simulink model "FullFMS_2026_02_25_V0_4_4"  (R2026a)
settings: Solver=FixedStepAuto  StopTime=inf  FixedStep=0.01  MaxStep=0.01  RelTol=1e-2
PreLoadFcn:
  | load("BUS_CONFIG.mat")
libraries: opcualib x8
(part 3 of 5)

== stateflow chart FullFMS_2026_02_25_V0_4_4/Chart ==
  state Variable_Declaration
    state VarDeclaration_20
      entry:
      %Actuators
      Actuators_20.F_22_Led_On;
      Actuators_20.F_22_Led_Off;
      Actuators_20.F_22_Conveyor;
      Actuators_20.F_24_Release_FB;
      Actuators_20.F_25_Release_FB;
      Actuators_20.F_26_Release_FB;
      Actuators_20.F_27_Release_FB;
      Actuators_20.F_28_Release_FB;
      Actuators_20.F_29_Release_FB;
      %Control
      Control_20.C_24_CartDel;
      Control_20.C_24_CRoute_Out;
      Control_20.C_24_Request;
      Control_20.C_24_CRoute_In;
      Control_20.C_25_CartDel;
      Control_20.C_25_CRoute_Out;
      Control_20.C_25_Request;
      Control_20.C_25_CRoute_In;
      Control_20.C_26_CartDel;
      Control_20.C_26_CRoute_Out;
      Control_20.C_26_Request;
      Control_20.C_26_CRoute_In;
      Control_20.C_27_CartDel;
      Control_20.C_27_CRoute_Out;
      Control_20.C_27_Request;
      Control_20.C_27_CRoute_In;
      Control_20.C_28_CartDel;
      Control_20.C_28_CRoute_Out;
      Control_20.C_28_Request;
      Control_20.C_28_CRoute_In;
      Control_20.C_29_CartDel;
      Control_20.C_29_CRoute_Out;
      Control_20.C_29_Request;
      Control_20.C_29_CRoute_In;
      %Sensors
      Sensors_20.O_20_On;
      Sensors_20.O_20_Off;
      Sensors_20.O_20_Controler_On;
      Sensors_20.O_24_Cart_Stat;
      Sensors_20.O_24_Cart_Next;
      Sensors_20.O_24_Optic;
      Sensors_20.O_24_Count;
      Sensors_20.O_24_Pist_Bck;
      Sensors_20.O_25_Cart_Stat;
      Sensors_20.O_25_Cart_Next;
      Sensors_20.O_25_Optic;
      Sensors_20.O_25_Count;
      Sensors_20.O_25_Pist_Bck;
      Sensors_20.O_26_Cart_Stat;
      Sensors_20.O_26_Cart_Next;
      Sensors_20.O_26_Optic;
      Sensors_20.O_26_Count;
      Sensors_20.O_26_Pist_Bck;
      Sensors_20.O_27_Cart_Stat;
      Sensors_20.O_27_Cart_Next;
      Sensors_20.O_27_Optic;
      Sensors_20.O_27_Count;
      Sensors_20.O_27_Pist_Bck;
      Sensors_20.O_28_Cart_Stat;
      Sensors_20.O_28_Cart_Next;
      Sensors_20.O_28_Optic;
      Sensors_20.O_28_Count;
      Sensors_20.O_28_Pist_Bck;
      Sensors_20.O_29_Cart_Stat;
      Sensors_20.O_29_Cart_Next;
      Sensors_20.O_29_Optic;
      Sensors_20.O_29_Count;
      Sensors_20.O_29_Pist_Bck;
    state VarDeclaration_30
      entry:
      %Actuators
      Actuators_30.F_33_Led_Start;
      Actuators_30.F_33_Led_Reset;
      Actuators_30.F_33_Led_Extra1;
      Actuators_30.F_33_Led_Extra2;
      Actuators_30.F_33_Spring_Cyl;
      Actuators_30.F_33_Cover_Cyl;
      %AS-i
      AS_i_30.A_34_Request;
      AS_i_30.A_34_No_Cart;
      AS_i_30.A_34_Cart_Full;
      AS_i_30.A_34_CRoute_Out;
      AS_i_30.A_32_RoboCartID;
      AS_i_30.A_34_Cart_Stat;
      AS_i_30.A_34_Cart_Next;
      AS_i_30.A_34_Optic;
      AS_i_30.A_34_Count;
      AS_i_30.A_34_Pist_Bck;
      AS_i_30.A_34_Release_FB;
      AS_i_30.A_34_CRoute_In;
      %Control
      Control_30.C_30_Robot1;
      Control_30.C_30_Robot2;
      Control_30.C_35_Part_Del;
      %Sensors
      Sensors_30.O_31_Start;
      Sensors_30.O_31_Stop;
      Sensors_30.O_31_Reset;
      Sensors_30.O_31_Part_in_Claw;
      Sensors_30.O_31_Orientation;
      Sensors_30.O_32_Sp_Cyl_Bck;
      Sensors_30.O_32_Sp_Cyl_Fwd;
      Sensors_30.O_32_Co_Cyl_Bck;
      Sensors_30.O_32_Co_Cyl_Fwd;
      Sensors_30.O_32_Sp_PickUp;
      Sensors_30.O_32_Co_PickUp;
      Sensors_30.O_32_CoMag_Empty;
    state VarDeclaration_40
      entry:
      %Actuators
      Actuators_40.F_43_Led_Start;
      Actuators_40.F_43_Led_Reset;
      Actuators_40.F_43_Led_Extra1;
      Actuators_40.F_43_Led_Extra2;
      Actuators_40.F_43_Panel_O4;
      Actuators_40.F_43_Panel_O5;
      Actuators_40.F_43_Panel_O6;
      Actuators_40.F_43_Panel_O7;
      %AS-i
      AS_i_40.A_44_Request;
      AS_i_40.A_44_No_Cart;
      AS_i_40.A_44_Cart_Full;
      AS_i_40.A_44_CRoute_Out;
      AS_i_40.A_43_StorCartID;
      AS_i_40.A_44_Cart_Stat;
      AS_i_40.A_44_Cart_Next;
      AS_i_40.A_44_Optic;
      AS_i_40.A_44_Count;
      AS_i_40.A_44_Pist_Bck;
      AS_i_40.A_44_Release_FB;
      AS_i_40.A_44_CRoute_In;
      %Control
      Control_40.C_45_Initialization;
      Control_40.C_42_Profibus;
      Control_40.C_45_Start;
      Control_40.C_45_StorePart;
      Control_40.C_45_RetrievePart;
      %Sensors
      Sensors_40.O_41_Start;
      Sensors_40.O_41_Stop;
      Sensors_40.O_41_Key_Pos;
      Sensors_40.O_41_Reset;
      Sensors_40.O_41_Panel_I4;
      Sensors_40.O_41_Panel_I5;
      Sensors_40.O_41_Panel_I6;
      Sensors_40.O_41_Panel_I7;
    state VarDeclaration_50
      entry:
      %Actuators
      Actuators_50.F_52_Claw_2_Del;
      Actuators_50.F_52_Claw_2_Cart;
      Actuators_50.F_52_Claw_Down;
      Actuators_50.F_52_Close_Claw;
      Actuators_50.F_53_Led_Start;
      Actuators_50.F_53_Led_Reset;
      Actuators_50.F_53_Led_Extra1;
      Actuators_50.F_53_Led_Extra2;
      Actuators_50.F_53_Panel_O4;
      Actuators_50.F_53_Panel_O5;
      Actuators_50.F_53_Panel_O6;
      Actuators_50.F_53_Panel_O7;
      %AS-i
      AS_i_50.A_54_Request;
      AS_i_50.A_54_No_Cart;
      AS_i_50.A_54_Cart_Full;
      AS_i_50.A_54_CRoute_Out;
      AS_i_50.A_53_SortCartID;
      AS_i_50.A_54_Cart_Stat;
      AS_i_50.A_54_Cart_Next;
      AS_i_50.A_54_Optic;
      AS_i_50.A_54_Count;
      AS_i_50.A_54_Pist_Bck;
      AS_i_50.A_54_Release_FB;
      AS_i_50.A_54_CRoute_In;
      %Control
      Control_50.C_55_Initialization;
      Control_50.C_55_PD_Sort;
      Control_50.C_52_Profibus;
      Control_50.C_55_Start;
      Control_50.C_55_Cart2Del;
      %Sensors
      Sensors_50.O_50_Part_Reserve;
      Sensors_50.O_50_Claw_Cart;
      Sensors_50.O_50_Claw_Del;
      Sensors_50.O_50_Claw_Reserve;
      Sensors_50.O_50_Claw_Low;
      Sensors_50.O_50_Claw_High;
      Sensors_50.O_50_Part_in_Claw;
      Sensors_50.O_51_Start;
      Sensors_50.O_51_Stop;
      Sensors_50.O_51_Key_Pos;
      Sensors_50.O_51_Reset;
      Sensors_50.O_51_Panel_I4;
      Sensors_50.O_51_Panel_I5;
      Sensors_50.O_51_Panel_I6;
      Sensors_50.O_51_Panel_I7;
    state VarDeclaration_60
      entry:
      %Actuators
      Actuators_60.F_62_Conveyor;
      Actuators_60.F_62_P1;
      Actuators_60.F_62_P2;
      Actuators_60.F_62_Identify;
      Actuators_60.F_63_Led_Start;
      Actuators_60.F_63_Led_Reset;
      Actuators_60.F_63_Led_Extra1;
      Actuators_60.F_63_Led_Extra2;
      Actuators_60.F_63_Panel_O4;
      Actuators_60.F_63_Panel_O5;
      Actuators_60.F_63_Panel_O6;
      Actuators_60.F_63_Panel_O7;
      %Control
      Control_60.C_65_Initialization;
      Control_60.C_65_ID_1;
      Control_60.C_65_ID_2;
      Control_60.C_65_Part_Sorted;
      Control_60.C_62_Profibus;
      Control_60.C_65_RBS_Output;
      Control_60.C_65_RSB_Output;
      Control_60.C_65_BRS_Output;
      Control_60.C_65_BSR_Output;
      Control_60.C_65_SRB_Output;
      Control_60.C_65_SBR_Output;
      %Sensors
      Sensors_60.O_60_SPart;
      Sensors_60.O_60_SInd;
      Sensors_60.O_60_SPhoto;
      Sensors_60.O_60_Part_Pass;
      Sensors_60.O_60_SL1_Bck;
      Sensors_60.O_60_SL1_Fwd;
      Sensors_60.O_60_SL2_Bck;
      Sensors_60.O_60_SL2_Fwd;
      Sensors_60.O_61_Start;
      Sensors_60.O_61_Stop;
      Sensors_60.O_61_Key_Pos;
      Sensors_60.O_61_Reset;
      Sensors_60.O_61_Panel_I4;
      Sensors_60.O_61_Panel_I5;
      Sensors_60.O_61_Panel_I6;
      Sensors_60.O_61_Panel_I7;
    state VarDeclaration_70
      entry:
      %Actuators
      Actuators_70.F_72_Elev_Down;
      Actuators_70.F_72_Elev_Up;
      Actuators_70.F_72_Eject_Part;
      Actuators_70.F_72_Air_On;
      Actuators_70.F_73_Led_Start;
      Actuators_70.F_73_Led_Reset;
      Actuators_70.F_73_Led_Extra1;
      Actuators_70.F_73_Led_Extra2;
      Actuators_70.F_73_Panel_O4;
      Actuators_70.F_73_Panel_O5;
      Actuators_70.F_73_Panel_O6;
      Actuators_70.F_73_Panel_O7;
      %AS-i
      AS_i_70.A_74_Request;
      AS_i_70.A_74_No_Cart;
      AS_i_70.A_74_Cart_Full;
      AS_i_70.A_74_CRoute_Out;
      AS_i_70.A_74_CRoute_In80;
      AS_i_70.A_73_TestCartID;
      AS_i_70.A_74_Cart_Stat;
      AS_i_70.A_74_Cart_Next;
      AS_i_70.A_74_Optic;
      AS_i_70.A_74_Count;
      AS_i_70.A_74_Pist_Bck;
      AS_i_70.A_74_Release_FB;
      AS_i_70.A_74_CRoute_In;
      %Control
      Control_70.C_75_Initialization;
      Control_70.C_75_ID_Delivery1;
      Control_70.C_75_ID_Delivery2;
      Control_70.C_75_Part_Del;
      Control_70.C_75_RQ_Part_Del;
      Control_70.C_75_RQ_Wrong;
      Control_70.C_75_Identified80;
      Control_70.C_75_Requested80;
      Control_70.C_72_Profibus;
      Control_70.C_75_RQ_Delivery1;
      Control_70.C_75_RQ_Delivery2;
      Control_70.C_75_Identified;
      Control_70.C_75_Requested;
      %Sensors
      Sensors_70.O_70_SInductive;
      Sensors_70.O_70_SPart;
      Sensors_70.O_70_SStation;
      Sensors_70.O_70_SPart_Height;
      Sensors_70.O_70_Elev_High;
      Sensors_70.O_70_Elev_Low;
      Sensors_70.O_70_Pist_Bck;
      Sensors_70.O_71_Start;
      Sensors_70.O_71_Stop;
      Sensors_70.O_71_Key_Pos;
      Sensors_70.O_71_Reset;
      Sensors_70.O_71_Panel_I4;
      Sensors_70.O_71_Panel_I5;
      Sensors_70.O_71_Panel_I6;
      Sensors_70.O_71_Panel_I7;
    state VarDeclaration_80
      entry:
      %Actuators
      Actuators_80.F_82_Pist_Adv;
      Actuators_80.F_82_Suction_On;
      Actuators_80.F_82_Suction_Off;
      Actuators_80.F_82_Arm_2_Del;
      Actuators_80.F_82_Arm_2_Mag;
      Actuators_80.F_83_Led_Start;
      Actuators_80.F_83_Led_Reset;
      Actuators_80.F_83_Led_Extra1;
      Actuators_80.F_83_Led_Extra2;
      Actuators_80.F_83_Panel_O4;
      Actuators_80.F_83_Panel_O5;
      Actuators_80.F_83_Panel_O6;
      Actuators_80.F_83_Panel_O7;
      %Control
      Control_80.C_85_Initialization;
      Control_80.C_85_Part_Del;
      Control_80.C_85_Part_Mag;
      Control_80.C_86_Mag_Parts;
      Control_80.C_87_RQ_MParts;
      Control_80.C_82_Profibus;
      Control_80.C_83_RQ_Parts;
      Control_80.C_85_Start;
      Control_80.C_85_Single;
      Control_80.C_85_Continuous;
      Control_80.C_85_Counted;
      %Sensors
      Sensors_80.O_80_Mag_Full;
      Sensors_80.O_80_Pist_Bck;
      Sensors_80.O_80_Pist_Fwd;
      Sensors_80.O_80_Part_Stuck;
      Sensors_80.O_80_Arm_Mag;
      Sensors_80.O_80_Arm_Del;
      Sensors_80.O_80_Mag_Empty;
      Sensors_80.O_81_Start;
      Sensors_80.O_81_Stop;,
      Sensors_80.O_81_Key_Pos;
      Sensors_80.O_81_Reset;
      Sensors_80.O_81_Panel_I4;
      Sensors_80.O_81_Panel_I5;
      Sensors_80.O_81_Panel_I6;
      Sensors_80.O_81_Panel_I7;
    state VarDeclaration_90
      entry:
      %Actuators
      Actuators_90.F_92_Claw_2_Cart;
      Actuators_90.F_92_Claw_2_Del;
      Actuators_90.F_92_Claw_Down;
      Actuators_90.F_92_Close_Claw;
      Actuators_90.F_93_Led_Start;
      Actuators_90.F_93_Led_Reset;
      Actuators_90.F_93_Led_Extra1;
      Actuators_90.F_93_Led_Extra2;
      Actuators_90.F_93_Panel_O4;
      Actuators_90.F_93_Panel_O5;
      Actuators_90.F_93_Panel_O6;
      Actuators_90.F_93_Panel_O7;
      %AS-i
      AS_i_90.A_94_Request;
      AS_i_90.A_94_No_Cart;
      AS_i_90.A_94_Cart_Full;
      AS_i_90.A_94_CRoute_Out;
      AS_i_90.A_93_ProcCartID;
      AS_i_90.A_94_Cart_Stat;
      AS_i_90.A_94_Cart_Next;
      AS_i_90.A_94_Optic;
      AS_i_90.A_94_Count;
      AS_i_90.A_94_Pist_Bck;
      AS_i_90.A_94_Release_FB;
      AS_i_90.A_94_CRoute_In;
      %Control
      Control_90.C_95_Initialization;
      Control_90.C_95_PD_Proc;
      Control_90.C_95_PD_Cart;
      Control_90.C_92_Profibus;
      Control_90.C_95_Start;
      Control_90.C_95_Cart2Del;
      Control_90.C_95_Del2Cart;
      %Sensors
      Sensors_90.O_90_Part_Reserve;
      Sensors_90.O_90_Claw_Del;
      Sensors_90.O_90_Claw_Cart;
      Sensors_90.O_90_Claw_Reserve;
      Sensors_90.O_90_Claw_Low;
      Sensors_90.O_90_Claw_High;
      Sensors_90.O_90_Part_in_Claw;
      Sensors_90.O_91_Start;
      Sensors_90.O_91_Stop;
      Sensors_90.O_91_Key_Pos;
      Sensors_90.O_91_Reset;
      Sensors_90.O_91_Panel_I4;
      Sensors_90.O_91_Panel_I5;
      Sensors_90.O_91_Panel_I6;
      Sensors_90.O_91_Panel_I7;
    state VarDeclaration_100
      entry:
      %Actuators
      Actuators_100.F_102_Drill_On;
      Actuators_100.F_102_RT_On;
      Actuators_100.F_102_Drill_Down;
      Actuators_100.F_102_Drill_Up;
      Actuators_100.F_102_Drill_Pin;
      Actuators_100.F_102_Test_Pin;
      Actuators_100.F_103_Led_Start;
      Actuators_100.F_103_Led_Reset;
      Actuators_100.F_103_Led_Extra1;
      Actuators_100.F_103_Led_Extra2;
      Actuators_100.F_103_Panel_O4;
      Actuators_100.F_103_Panel_O5;
      Actuators_100.F_103_Panel_O6;
      Actuators_100.F_103_Panel_O7;
      %Control
      Control_100.C_105_Initialization;
      Control_100.C_105_Part_ready;
      Control_100.C_105_Test_Ok;
      Control_100.C_105_Test_Fail;
      Control_100.C_106_RT_Counter;
      Control_100.C_102_Profibus;
      Control_100.C_103_RQ_Turns;
      Control_100.C_105_Start;
      Control_100.C_105_Test;
      Control_100.C_105_TestDrill;
      Control_100.C_105_Rotation;
      %Sensors
      Sensors_100.O_100_PInit_Pos;
      Sensors_100.O_100_PDrill_Pos;
      Sensors_100.O_100_PTest_Pos;
      Sensors_100.O_100_SDrill_High;
      Sensors_100.O_100_SDrill_Low;
      Sensors_100.O_100_RT_Sensor;
      Sensors_100.O_100_PTest_Ok;
      Sensors_100.O_101_Start;
      Sensors_100.O_101_Stop;
      Sensors_100.O_101_Key_Pos;
      Sensors_100.O_101_Reset;
      Sensors_100.O_101_Panel_I4;
      Sensors_100.O_101_Panel_I5;
      Sensors_100.O_101_Panel_I6;
      Sensors_100.O_101_Panel_I7;
    (default) -> VarDeclaration_20
    VarDeclaration_60 -> VarDeclaration_70
    VarDeclaration_30 -> VarDeclaration_40
    VarDeclaration_40 -> VarDeclaration_50
    VarDeclaration_70 -> VarDeclaration_80
    VarDeclaration_80 -> VarDeclaration_90
    VarDeclaration_50 -> VarDeclaration_60
    VarDeclaration_90 -> VarDeclaration_100
    VarDeclaration_20 -> VarDeclaration_30
  note: Sorting [60]
  state BRS Output
    state ArmToMagazine1
      entry:
      Status2c_14 = false;
      during:
      Actuators_80.F_82_Suction_Off;
      Actuators_80.F_82_Arm_2_Mag;
      Actuators_80.F_83_Led_Extra1;
      Control_80.C_85_Part_Del;
      if ~Actuators_80.F_82_Suction_Off && ...
      Actuators_80.F_82_Arm_2_Mag && ...
      Actuators_80.F_83_Led_Extra1 && ...
      Control_80.C_85_Part_Del
      Status2c_14 = true;
      else
      Status2c_14 = false;
      end
    state ArmCloseDeliver3
      entry:
      Status2c_15 = false;
      during:
      Sensors_70.O_70_SStation;
      if Sensors_70.O_70_SStation
      Status2c_15 = true;
      else
      Status2c_15 = false;
      end
    state ArmArrives_Finish
      entry:
      Status2c_16 = false;
      during:
      Actuators_80.F_82_Arm_2_Mag;
      if ~Actuators_80.F_82_Arm_2_Mag;
      Status2c_16 = true;
      else
      Status2c_16 = false;
      end
    state ArmToMagazine
      entry:
      Status2c_8 = false;
      during:
      Actuators_80.F_82_Arm_2_Mag;
      if Actuators_80.F_82_Arm_2_Mag
      Status2c_8 = true;
      else
      Status2c_8 = false;
      end
    state ArmCloseDeliver1
      entry:
      Status2c_9 = false;
      during:
      Sensors_70.O_70_SStation;
      if Sensors_70.O_70_SStation
      Status2c_9 = true;
      else
      Status2c_9 = false;
      end
    state ArmArrives_PicksPart
      entry:
      Status2c_10 = false;
      during:
      Actuators_80.F_82_Suction_On;
      Actuators_80.F_82_Arm_2_Mag;
      if Actuators_80.F_82_Suction_On && ...
      ~Actuators_80.F_82_Arm_2_Mag
      Status2c_10 = true;
      else
      Status2c_10 = false;
      end
    state ArmToDelivery1
      entry:
      Status2c_11 = false;
      during:
      Actuators_80.F_82_Arm_2_Del
      if Actuators_80.F_82_Arm_2_Del
      Status2c_11 = true;
      else
      Status2c_11 = false;
      end
    state ArmCloseDelivery2
      entry:
      Status2c_12 = false;
      during:
      Sensors_70.O_70_SStation;
      if Sensors_70.O_70_SStation
      Status2c_12 = true;
      else
      Status2c_12 = false;
      end
    state ArmArrives_DeliversPart
      entry:
      Status2c_13 = false;
      during:
      Actuators_80.F_82_Suction_On;
      Actuators_80.F_82_Suction_Off;
      Actuators_80.F_82_Arm_2_Del;
      if ~Actuators_80.F_82_Suction_On && ...
      Actuators_80.F_82_Suction_Off && ...
      ~Actuators_80.F_82_Arm_2_Del
      Status2c_13 = true;
      else
      Status2c_13 = false;
      end
    state PartDel_CheckLoop
      entry:
      LoopDistCont = false;
      during:
      Control_80.C_85_Part_Del
      Control_80.C_87_RQ_MParts
      if Control_80.C_85_Part_Del && ...
      Control_80.C_87_RQ_MParts == 0
      LoopDistCont = true;
      else
      LoopDistCont = false;
      end
    state InitialCondition
      entry:
      Status2c_1 = false;
      during:
      Control_80.C_85_Initialization;
      Control_80.C_86_Mag_Parts;
      Control_80.C_82_Profibus;
      Control_80.C_85_Continuous;
      Sensors_80.O_80_Arm_Mag;
      Sensors_80.O_81_Key_Pos;
      if Control_80.C_85_Initialization&& ...
      Control_80.C_86_Mag_Parts ~= 0 && ...
      Control_80.C_82_Profibus && ...
      Control_80.C_85_Continuous && ...
      Sensors_80.O_80_Arm_Mag && ...
      Sensors_80.O_81_Key_Pos
      Status2c_1 = true;
      else
      Status2c_1 = false;
      end
    state ArmToDelivery
      entry:
      Status2c_2 = false;
      during:
      Actuators_80.F_82_Arm_2_Del
      if Actuators_80.F_82_Arm_2_Del
      Status2c_2 = true;
      else
      Status2c_2 = false;
      end
    state ArmCloseDelivery
      entry:
      Status2c_3 = false;
      during:
      Sensors_70.O_70_SStation;
      if Sensors_70.O_70_SStation
      Status2c_3 = true;
      else
      Status2c_3 = false;
      end
    state ArmArrives_FeedsPart
      entry:
      Status2b_4 = false;
      during:
      Actuators_80.F_82_Pist_Adv;
      Actuators_80.F_82_Arm_2_Del;
      if Actuators_80.F_82_Pist_Adv && ...
      ~Actuators_80.F_82_Arm_2_Del
      Status2b_4 = true;
      else
      Status2b_4 = false;
      end
    state PistonStartsMoveForward
      entry:
      Status2c_5 = false;
      during:
      Sensors_80.O_80_Pist_Bck;
      if ~Sensors_80.O_80_Pist_Bck
      Status2c_5 = true;
      else
      Status2c_5 = false;
      end
    state PartFed
      entry:
      Status2c_6 = false;
      during:
      Actuators_80.F_82_Pist_Adv;
      if ~Actuators_80.F_82_Pist_Adv
      Status2c_6 = true;
      else
      Status2c_6 = false;
      end
    state PistonStartsMoveBackward
      entry:
      Status2c_7 = false;
      during:
      Sensors_80.O_80_Pist_Fwd;
      if ~Sensors_80.O_80_Pist_Fwd
      Status2c_7 = true;
      else
      Status2c_7 = false;
      end
    state T1
      during:
      Control_80.C_85_Part_Del
      Actuators_80.F_83_Led_Extra1
    BRS.InitialCondition -> BRS.ArmToDelivery : [Sensors_80.O_81_Start == true | ...
        | Control_80.C_85_Start == true | ...
        | Control_70.C_75_RQ_Wrong == true | ...
        | (AS_i_70.A_74_CRoute_In80 == true && Sensors_80.O_81_Key_Pos == true) ]
    BRS.ArmArrives_FeedsPart -> BRS.PistonStartsMoveForward : [Status2b_4 == true]
    BRS.PartDel_CheckLoop -> BRS.ArmToMagazine1 [order 2] : [LoopDistCont == false]
    BRS.ArmCloseDeliver3 -> BRS.ArmArrives_Finish : [Sensors_80.O_80_Arm_Mag == true && ...
        | Status2c_15 == true]
    BRS.ArmCloseDelivery2 -> BRS.ArmArrives_DeliversPart : [Sensors_80.O_80_Arm_Del == true && ...
        | Status2c_12 == true]
    BRS.ArmCloseDelivery -> BRS.ArmArrives_FeedsPart : [Sensors_80.O_80_Arm_Del == true && ...
        | Status2c_3 == true]
    BRS.PistonStartsMoveForward -> BRS.PartFed : [Sensors_80.O_80_Pist_Fwd == true && ...
        | Status2c_5 == true]
    BRS.ArmArrives_DeliversPart -> BRS.PartDel_CheckLoop : [Sensors_80.O_80_Part_Stuck == false && ...
        | Status2c_13 == true]
    BRS.ArmToMagazine1 -> BRS.ArmCloseDeliver3 : [Sensors_80.O_80_Arm_Del == false &&...
        | Status2c_14 == true]
    BRS.ArmArrives_PicksPart -> BRS.ArmToDelivery1 : [Sensors_80.O_80_Part_Stuck == true && ...
        | Status2c_10 == true]
    BRS.PistonStartsMoveBackward -> BRS.ArmToMagazine : [Sensors_80.O_80_Pist_Bck == true && ...
        | Status2c_7 == true]
    BRS.ArmToDelivery -> BRS.ArmCloseDelivery : [Sensors_80.O_80_Arm_Mag == false &&...
        | Status2c_2 == true]
    BRS.ArmToMagazine -> BRS.ArmCloseDeliver1 : [Sensors_80.O_80_Arm_Del == false &&...
        | Status2c_8 == true]
    BRS.ArmCloseDeliver1 -> BRS.ArmArrives_PicksPart : [Sensors_80.O_80_Arm_Mag == true && ...
        | Status2c_9 == true]
    BRS.PartFed -> BRS.PistonStartsMoveBackward : [Status2c_6 == true]
    (default) -> BRS.InitialCondition
    BRS.ArmToDelivery1 -> BRS.ArmCloseDelivery2 : [Sensors_80.O_80_Arm_Mag == false &&...
        | Status2c_11 == true]
    (junction 2320) -> BRS.ArmArrives_FeedsPart
    (junction 2303) -> (junction 2320)
    BRS.PartDel_CheckLoop -> (junction 2308) [order 1] : [LoopDistCont == true]
    BRS.PartDel_CheckLoop -> BRS.T1 [order 3] : after(4,sec)
    (junction 2308) -> (junction 2303)
  state Start
    during:
    Control_20.C_24_Request
  note: Conveyor
  state CartToTesting
    state StartsProcess
      entry:
      Status1_2 = false;
      during:
      Actuators_20.F_22_Conveyor;
      AS_i_50.A_53_SortCartID;
      AS_i_50.A_54_Pist_Bck;
      AS_i_50.A_54_Release_FB;
      if Actuators_20.F_22_Conveyor && ...
      AS_i_50.A_53_SortCartID == 0 && ...
      AS_i_50.A_54_Pist_Bck && ...
      AS_i_50.A_54_Release_FB
      Status1_2 = true;
      else
      Status1_2 = false;
      end
    state CartStartsMoving
      entry:
      Status1_3 = false;
      during:
      Actuators_50.F_53_Led_Extra1;
      AS_i_50.A_54_No_Cart;
      AS_i_50.A_54_Cart_Stat;
      if Actuators_50.F_53_Led_Extra1 && ...
      AS_i_50.A_54_No_Cart && ...
      ~AS_i_50.A_54_Cart_Stat
      Status1_3 = true;
      else
      Status1_3 = false;
      end
    state CartGetsNearNextStation
      entry:
      Status1_4 = false;
      during:
      AS_i_50.A_54_Cart_Next;
      AS_i_50.A_54_Pist_Bck;
      AS_i_50.A_54_Release_FB;
      if AS_i_50.A_54_Cart_Next && ...
      ~AS_i_50.A_54_Pist_Bck & ...
      ~AS_i_50.A_54_Release_FB
      Status1_4 = true;
      else
      Status1_4 = false;
      end
    state DetectionofCartNumberinStation
      entry:
      Status1_5 = false;
      during:
      AS_i_70.A_73_TestCartID
      if AS_i_70.A_73_TestCartID ~= 0
      Status1_5 = true;
      else
      Status1_5 = false;
      end
    state CartPassesNextStation
      entry:
      Status1_6 = false;
      during:
      AS_i_50.A_54_Cart_Next;
      if ~AS_i_50.A_54_Cart_Next;
      Status1_6 = true;
      else
      Status1_6 = false;
      end
    state CartArrivesinNextStation
      entry:
      Status1_7 = false;
      during:
      Control_20.C_24_CartDel;
      Actuators_70.F_73_Led_Extra1;
      AS_i_70.A_74_No_Cart;
      AS_i_70.A_74_Cart_Stat;
      AS_i_70.A_74_CRoute_In;
      if Control_20.C_24_CartDel;
      ~Actuators_70.F_73_Led_Extra1;
      ~AS_i_70.A_74_No_Cart;
      AS_i_70.A_74_Cart_Stat;
      AS_i_70.A_74_CRoute_In;
      Status1_7 = true;
      else
      Status1_7 = false;
      end
    state InitialCondition
      entry:
      Status1_1 = false;
      during:
      Actuators_20.F_22_Conveyor;
      AS_i_50.A_53_SortCartID;
      AS_i_50.A_54_Pist_Bck;
      AS_i_50.A_54_Release_FB;
      if ~Actuators_20.F_22_Conveyor && ...
      ~AS_i_50.A_53_SortCartID ~= 0 && ...
      ~AS_i_50.A_54_Pist_Bck && ...
      ~AS_i_50.A_54_Release_FB
      Status1_1 = true;
      else
      Status1_1 = false;
      end
    state T1
      during:
      Control_20.C_24_Request
    state T3
      during:
      Control_20.C_24_CartDel
    state T2
      during:
      AS_i_70.A_74_CRoute_In
    CartToTesting.CartStartsMoving -> CartToTesting.CartGetsNearNextStation : [Sensors_20.O_29_Cart_Next == true && ...
        | Status1_3 == true]
    CartToTesting.CartPassesNextStation -> CartToTesting.CartArrivesinNextStation : [Sensors_20.O_24_Cart_Stat == true && ...
        | Status1_6 == true]
    (default) -> CartToTesting.InitialCondition
    CartToTesting.InitialCondition -> CartToTesting.StartsProcess : [Control_20.C_24_Request == true && ...
        |  Status1_1 == true]
    CartToTesting.CartGetsNearNextStation -> CartToTesting.DetectionofCartNumberinStation : [Sensors_20.O_29_Count == true && ...
        | Status1_4 == true]
    CartToTesting.DetectionofCartNumberinStation -> CartToTesting.CartPassesNextStation : [Sensors_20.O_29_Cart_Next == false && ...
        | Status1_5 == true]
    CartToTesting.StartsProcess -> CartToTesting.CartStartsMoving [order 1] : [Sensors_20.O_29_Cart_Stat == false && ...
        |  Status1_2 == true]
    CartToTesting.StartsProcess -> CartToTesting.T1 [order 2] : [after(2, sec)]
    CartToTesting.CartArrivesinNextStation -> (junction 582)
    (junction 582) -> CartToTesting.T3 [order 2] : [after(3,sec)]
    (junction 582) -> CartToTesting.T2 [order 1] : [after(2,sec)]
  state BSR Output
    state ArmToMagazine1
      entry:
      Status2c_14 = false;
      during:
      Actuators_80.F_82_Suction_Off;
      Actuators_80.F_82_Arm_2_Mag;
      Actuators_80.F_83_Led_Extra1;
      Control_80.C_85_Part_Del;
      if ~Actuators_80.F_82_Suction_Off && ...
      Actuators_80.F_82_Arm_2_Mag && ...
      Actuators_80.F_83_Led_Extra1 && ...
      Control_80.C_85_Part_Del
      Status2c_14 = true;
      else
      Status2c_14 = false;
      end
    state ArmCloseDeliver3
      entry:
      Status2c_15 = false;
      during:
      Sensors_70.O_70_SStation;
      if Sensors_70.O_70_SStation
      Status2c_15 = true;
      else
      Status2c_15 = false;
      end
    state ArmArrives_Finish
      entry:
      Status2c_16 = false;
      during:
      Actuators_80.F_82_Arm_2_Mag;
      if ~Actuators_80.F_82_Arm_2_Mag;
      Status2c_16 = true;
      else
      Status2c_16 = false;
      end
    state ArmToMagazine
      entry:
      Status2c_8 = false;
      during:
      Actuators_80.F_82_Arm_2_Mag;
      if Actuators_80.F_82_Arm_2_Mag
      Status2c_8 = true;
      else
      Status2c_8 = false;
      end
    state ArmCloseDeliver1
      entry:
      Status2c_9 = false;
      during:
      Sensors_70.O_70_SStation;
      if Sensors_70.O_70_SStation
      Status2c_9 = true;
      else
      Status2c_9 = false;
      end
    state ArmArrives_PicksPart
      entry:
      Status2c_10 = false;
      during:
      Actuators_80.F_82_Suction_On;
      Actuators_80.F_82_Arm_2_Mag;
      if Actuators_80.F_82_Suction_On && ...
      ~Actuators_80.F_82_Arm_2_Mag
      Status2c_10 = true;
      else
      Status2c_10 = false;
      end
    state ArmToDelivery1
      entry:
      Status2c_11 = false;
      during:
      Actuators_80.F_82_Arm_2_Del
      if Actuators_80.F_82_Arm_2_Del
      Status2c_11 = true;
      else
      Status2c_11 = false;
      end
    state ArmCloseDelivery2
      entry:
      Status2c_12 = false;
      during:
      Sensors_70.O_70_SStation;
      if Sensors_70.O_70_SStation
      Status2c_12 = true;
      else
      Status2c_12 = false;
      end
    state ArmArrives_DeliversPart
      entry:
      Status2c_13 = false;
      during:
      Actuators_80.F_82_Suction_On;
      Actuators_80.F_82_Suction_Off;
      Actuators_80.F_82_Arm_2_Del;
      if ~Actuators_80.F_82_Suction_On && ...
      Actuators_80.F_82_Suction_Off && ...
      ~Actuators_80.F_82_Arm_2_Del
      Status2c_13 = true;
      else
      Status2c_13 = false;
      end
    state PartDel_CheckLoop
      entry:
      LoopDistCont = false;
      during:
      Control_80.C_85_Part_Del
      Control_80.C_87_RQ_MParts
      if Control_80.C_85_Part_Del && ...
      Control_80.C_87_RQ_MParts == 0
      LoopDistCont = true;
      else
      LoopDistCont = false;
      end
    state InitialCondition
      entry:
      Status2c_1 = false;
      during:
      Control_80.C_85_Initialization;
      Control_80.C_86_Mag_Parts;
      Control_80.C_82_Profibus;
      Control_80.C_85_Continuous;
      Sensors_80.O_80_Arm_Mag;
      Sensors_80.O_81_Key_Pos;
      if Control_80.C_85_Initialization&& ...
      Control_80.C_86_Mag_Parts ~= 0 && ...
      Control_80.C_82_Profibus && ...
      Control_80.C_85_Continuous && ...
      Sensors_80.O_80_Arm_Mag && ...
      Sensors_80.O_81_Key_Pos
      Status2c_1 = true;
      else
      Status2c_1 = false;
      end
    state ArmToDelivery
      entry:
      Status2c_2 = false;
      during:
      Actuators_80.F_82_Arm_2_Del
      if Actuators_80.F_82_Arm_2_Del
      Status2c_2 = true;
      else
      Status2c_2 = false;
      end
    state ArmCloseDelivery
      entry:
      Status2c_3 = false;
      during:
      Sensors_70.O_70_SStation;
      if Sensors_70.O_70_SStation
      Status2c_3 = true;
      else
      Status2c_3 = false;
      end
    state ArmArrives_FeedsPart
      entry:
      Status2b_4 = false;
      during:
      Actuators_80.F_82_Pist_Adv;
      Actuators_80.F_82_Arm_2_Del;
      if Actuators_80.F_82_Pist_Adv && ...
      ~Actuators_80.F_82_Arm_2_Del
      Status2b_4 = true;
      else
      Status2b_4 = false;
      end
    state PistonStartsMoveForward
      entry:
      Status2c_5 = false;
      during:
      Sensors_80.O_80_Pist_Bck;
      if ~Sensors_80.O_80_Pist_Bck
      Status2c_5 = true;
      else
      Status2c_5 = false;
      end
    state PartFed
      entry:
      Status2c_6 = false;
      during:
      Actuators_80.F_82_Pist_Adv;
      if ~Actuators_80.F_82_Pist_Adv
      Status2c_6 = true;
      else
      Status2c_6 = false;
      end
    state PistonStartsMoveBackward
      entry:
      Status2c_7 = false;
      during:
      Sensors_80.O_80_Pist_Fwd;
      if ~Sensors_80.O_80_Pist_Fwd
      Status2c_7 = true;
      else
      Status2c_7 = false;
      end
    state T1
      during:
      Control_80.C_85_Part_Del
      Actuators_80.F_83_Led_Extra1
    BSR.InitialCondition -> BSR.ArmToDelivery : [Sensors_80.O_81_Start == true | ...
        | Control_80.C_85_Start == true | ...
        | Control_70.C_75_RQ_Wrong == true | ...
        | (AS_i_70.A_74_CRoute_In80 == true && Sensors_80.O_81_Key_Pos == true) ]
    BSR.ArmArrives_FeedsPart -> BSR.PistonStartsMoveForward : [Status2b_4 == true]
    BSR.PartDel_CheckLoop -> BSR.ArmToMagazine1 [order 2] : [LoopDistCont == false]
    BSR.ArmCloseDeliver3 -> BSR.ArmArrives_Finish : [Sensors_80.O_80_Arm_Mag == true && ...
        | Status2c_15 == true]
    BSR.ArmCloseDelivery2 -> BSR.ArmArrives_DeliversPart : [Sensors_80.O_80_Arm_Del == true && ...
        | Status2c_12 == true]
    BSR.ArmCloseDelivery -> BSR.ArmArrives_FeedsPart : [Sensors_80.O_80_Arm_Del == true && ...
        | Status2c_3 == true]
    BSR.PistonStartsMoveForward -> BSR.PartFed : [Sensors_80.O_80_Pist_Fwd == true && ...
        | Status2c_5 == true]
    BSR.ArmArrives_DeliversPart -> BSR.PartDel_CheckLoop : [Sensors_80.O_80_Part_Stuck == false && ...
        | Status2c_13 == true]
    BSR.ArmToMagazine1 -> BSR.ArmCloseDeliver3 : [Sensors_80.O_80_Arm_Del == false &&...
        | Status2c_14 == true]
    BSR.ArmArrives_PicksPart -> BSR.ArmToDelivery1 : [Sensors_80.O_80_Part_Stuck == true && ...
        | Status2c_10 == true]
    BSR.PistonStartsMoveBackward -> BSR.ArmToMagazine : [Sensors_80.O_80_Pist_Bck == true && ...
        | Status2c_7 == true]
    BSR.ArmToDelivery -> BSR.ArmCloseDelivery : [Sensors_80.O_80_Arm_Mag == false &&...
        | Status2c_2 == true]
    BSR.ArmToMagazine -> BSR.ArmCloseDeliver1 : [Sensors_80.O_80_Arm_Del == false &&...
        | Status2c_8 == true]
    BSR.ArmCloseDeliver1 -> BSR.ArmArrives_PicksPart : [Sensors_80.O_80_Arm_Mag == true && ...
        | Status2c_9 == true]
    BSR.PartFed -> BSR.PistonStartsMoveBackward : [Status2c_6 == true]
    (default) -> BSR.InitialCondition
    BSR.ArmToDelivery1 -> BSR.ArmCloseDelivery2 : [Sensors_80.O_80_Arm_Mag == false &&...
        | Status2c_11 == true]
    (junction 2276) -> BSR.ArmArrives_FeedsPart
    (junction 2259) -> (junction 2276)
    BSR.PartDel_CheckLoop -> (junction 2264) [order 1] : [LoopDistCont == true]
    BSR.PartDel_CheckLoop -> BSR.T1 [order 3] : after(4,sec)
    (junction 2264) -> (junction 2259)
  note: Testing Station [70]
  note: Distribution Station [80]
  state Identified_Delivery
    state Part_HeightSensor
      entry:
      Status3a_8 = false;
      during:
      Actuators_70.F_72_Eject_Part;
      Sensors_70.O_70_Pist_Bck;
      Sensors_70.O_70_SPart_Height
      if Actuators_70.F_72_Eject_Part && ...
      ~Sensors_70.O_70_Pist_Bck && ...
      ~Sensors_70.O_70_SPart_Height
      Status3a_8 = true
      else
      Status3a_8 = false
      end
    state Piston_Back
      entry:
      Status3a_10 = false;
      during:
      Actuators_70.F_72_Eject_Part
      if ~Actuators_70.F_72_Eject_Part
      Status3a_10 = true
      else
      Status3a_10 = false
      end
    state Elevator_StartsMovingDown
      entry:
      Status3a_11 = false;
      during:
      Actuators_70.F_72_Elev_Down;
      Actuators_70.F_72_Elev_Up;
      if Actuators_70.F_72_Elev_Down && ...
      ~Actuators_70.F_72_Elev_Up
      Status3a_11 = true
      else
      Status3a_11 = false
      end
    state Elevator_MiddleDown
      entry:
      Status3a_12 = false;
      during:
      Sensors_70.O_70_SStation;
      if ~Sensors_70.O_70_SStation
      Status3a_12 = true
      else
      Status3a_12 = false
      end
    state Elevator_InductiveDown
      entry:
      Status3a_13 = false;
      during:
      Sensors_70.O_70_SInductive;
      if ~Sensors_70.O_70_SInductive
      Status3a_13 = true
      else
      Status3a_13 = false
      end
    state Pushes_Part
      entry:
      Status3a_7 = false;
      during:
      Actuators_70.F_72_Eject_Part;
      Actuators_70.F_72_Air_On;
      Sensors_70.O_70_SPart;
      if Actuators_70.F_72_Eject_Part && ...
      Actuators_70.F_72_Air_On && ...
      ~Sensors_70.O_70_SPart
      Status3a_7 = true
      else
      Status3a_7 = false
      end
    state InitialCondition
      entry:
      Status3a_1 = false;
      during:
      AS_i_70.A_74_Cart_Full;
      Control_70.C_75_Initialization;
      Control_70.C_72_Profibus;
      Control_70.C_75_Identified;
      Sensors_70.O_70_SPart;
      Sensors_70.O_71_Key_Pos;
      if ~AS_i_70.A_74_Cart_Full && ...
      Control_70.C_75_Initialization && ...
      Control_70.C_72_Profibus && ...
      Control_70.C_75_Identified && ...
      ~Sensors_70.O_70_SPart && ...
      Sensors_70.O_71_Key_Pos
      Status3a_1 = true;
      else
      Status3a_1 = false;
      end
    state Part_Arrives
      entry:
      Status3a_2 = false;
      during:
      Control_70.C_75_ID_Delivery2;
      Sensors_70.O_70_SInductive;
      Sensors_70.O_70_SPart;
      Sensors_80.O_80_Arm_Mag;
      if Sensors_70.O_70_SPart && ...
      ((Sensors_70.O_70_SInductive && ...
      Control_70.C_75_ID_Delivery2) | ...
      (~Sensors_70.O_70_SInductive && ...
      ~Control_70.C_75_ID_Delivery2)) && ...
      ~Sensors_80.O_80_Arm_Mag
      Status3a_2 = true;
      else
      Status3a_2 =false;
      end
    state Elevator_Up
      entry:
      Status3a_3 = false;
      during:
      Actuators_70.F_72_Elev_Up;
      if Actuators_70.F_72_Elev_Up
      Status3a_3 = true
      else
      Status3a_3 = false
      end
    state Elevator_StartsMovingUp
      entry:
      Status3a_4 = false;
      during:
      Sensors_70.O_70_SInductive;
      if ~Sensors_70.O_70_SInductive
      Status3a_4 = true
      else
      Status3a_4 = false
      end
    state Elevator_MiddleUp
      entry:
      Status3a_5 = false;
      during:
      Sensors_70.O_70_SStation;
      if ~Sensors_70.O_70_SStation
      Status3a_5 = true
      else
      Status3a_5 = false
      end
    state Elevator_High_Identify_Part
      entry:
      Status3a_6 = false;
      during:
      MetalicPart;
      Control_70.C_75_ID_Delivery1;
      Control_70.C_75_ID_Delivery2;
      Sensors_70.O_70_SPart_Height;
      if MetalicPart && ...
      Control_70.C_75_ID_Delivery2 && ...
      ~Control_70.C_75_ID_Delivery1;
      Status3a_6 = true
      end
      if ~MetalicPart && ...
      Control_70.C_75_ID_Delivery1 && ...
      ((Sensors_70.O_70_SPart_Height && ...
      Control_70.C_75_ID_Delivery2) | ...
      (~Sensors_70.O_70_SPart_Height && ...
      ~Control_70.C_75_ID_Delivery2))
      Status3a_6=true
      end
    state Elevator_Down
      entry:
      Status3a_14 = false;
      during:
      AS_i_70.A_74_CRoute_Out;
      Actuators_70.F_72_Elev_Down;
      Control_70.C_75_Part_Del;
      if AS_i_70.A_74_CRoute_Out && ...
      ~Actuators_70.F_72_Elev_Down&& ...
      Control_70.C_75_Part_Del
      Status3a_14 = true
      else
      Status3a_14 = false
      end
    state Part_ArrivesAtCart
      entry:
      Status3a_9 = false;
      during:
      AS_i_70.A_74_Cart_Full;
      AS_i_70.A_74_Optic;
      Actuators_70.F_72_Air_On;
      Actuators_70.F_73_Led_Extra2
      if AS_i_70.A_74_Optic && ...
      AS_i_70.A_74_Cart_Full && ...
      ~Actuators_70.F_72_Air_On && ...
      Actuators_70.F_73_Led_Extra2;
      Status3a_9 = true
      else
      Status3a_9 = false
      end
    state End_Process
      entry:
      Status3a_15 = false;
      during:
      AS_i_70.A_74_CRoute_Out;
      if  ~AS_i_70.A_74_CRoute_Out;
      Status3a_15 = true
      else
      Status3a_15 = false
      end
    state Metalic_Identify
      entry:
      MetalicPart = false;
      during:
      Sensors_70.O_70_SInductive;
      if Sensors_70.O_70_SInductive
      MetalicPart = true
      else
      MetalicPart = false
      end
    (default) -> Identified_Delivery.InitialCondition
    Identified_Delivery.Elevator_StartsMovingDown -> Identified_Delivery.Elevator_MiddleDown : [Status3a_11 == true && ...
        | Sensors_70.O_70_SStation == true]
    Identified_Delivery.Piston_Back -> Identified_Delivery.Elevator_StartsMovingDown : [Status3a_10 == true && ...
        | Sensors_70.O_70_Pist_Bck == true]
    Identified_Delivery.Elevator_MiddleDown -> Identified_Delivery.Elevator_InductiveDown : [Status3a_12 == true && ...
        | Sensors_70.O_70_SInductive == true]
    Identified_Delivery.Part_Arrives -> Identified_Delivery.Elevator_Up : [Status3a_2 == true && ...
        | Sensors_80.O_80_Arm_Mag == true ]
    Identified_Delivery.Elevator_High_Identify_Part -> Identified_Delivery.Pushes_Part : [Status3a_6 == true && ...
        | after (2,sec)]
    Identified_Delivery.Pushes_Part -> Identified_Delivery.Part_HeightSensor : [Status3a_7 == true && ...
        | Sensors_70.O_70_Pist_Bck == false]
    Identified_Delivery.Elevator_Up -> Identified_Delivery.Elevator_StartsMovingUp : [Status3a_3 == true && ...
        | Sensors_70.O_70_SInductive == true ]
    Identified_Delivery.Elevator_InductiveDown -> Identified_Delivery.Elevator_Down : [Status3a_13 == true && ...
        | Sensors_70.O_70_Elev_Low == true]
    Identified_Delivery.Part_HeightSensor -> (junction 1354)
    (junction 1354) -> Identified_Delivery.Piston_Back [order 1] : [Status3a_8 == true && ...
        | after (2,sec)]
    Identified_Delivery.Elevator_StartsMovingUp -> Identified_Delivery.Elevator_MiddleUp : [Status3a_4 == true && ...
        | Sensors_70.O_70_SStation == true]
    Identified_Delivery.Elevator_MiddleUp -> Identified_Delivery.Elevator_High_Identify_Part : [Status3a_5 == true && ...
        | Sensors_70.O_70_Elev_High == true]
    Identified_Delivery.InitialCondition -> (junction 1348) : [Status3a_1 == true && ...
        | Sensors_70.O_70_SPart == true]
    (junction 1348) -> Identified_Delivery.Part_Arrives [order 1]
    (junction 1354) -> (junction 1356) [order 2] : [Status3a_8 == true && ...
        | AS_i_70.A_74_Optic == true]
    (junction 1348) -> (junction 1350) [order 2]
    Identified_Delivery.Elevator_Down -> Identified_Delivery.End_Process : after (2,sec)
    (junction 1356) -> Identified_Delivery.Part_ArrivesAtCart
    (junction 1350) -> Identified_Delivery.Metalic_Identify
  state Distribution_Single
    state PistonStartsMoveBackward
      entry:
      Status2a_7 = false;
      during:
      Sensors_80.O_80_Pist_Fwd;
      if ~Sensors_80.O_80_Pist_Fwd
      Status2a_7 = true;
      else
      Status2a_7 = false;
      end
    state PartFed
      entry:
      Status2a_6 = false;
      during:
      Actuators_80.F_82_Pist_Adv;
      if ~Actuators_80.F_82_Pist_Adv
      Status2a_6 = true;
      else
      Status2a_6 = false;
      end
    state ArmToMagazine
      entry:
      Status2a_8 = false;
      during:
      Actuators_80.F_82_Arm_2_Mag;
      if Actuators_80.F_82_Arm_2_Mag
      Status2a_8 = true;
      else
      Status2a_8 = false;
      end
    state ArmCloseDeliver1
      entry:
      Status2a_9 = false;
      during:
      Sensors_70.O_70_SStation;
      if Sensors_70.O_70_SStation
      Status2a_9 = true;
      else
      Status2a_9 = false;
      end
    state ArmArrives_PicksPart
      entry:
      Status2a_10 = false;
      during:
      Actuators_80.F_82_Suction_On;
      Actuators_80.F_82_Arm_2_Mag;
      if Actuators_80.F_82_Suction_On && ...
      ~Actuators_80.F_82_Arm_2_Mag
      Status2a_10 = true;
      else
      Status2a_10 = false;
      end
    state ArmToDelivery1
      entry:
      Status2a_11 = false;
      during:
      Actuators_80.F_82_Arm_2_Del
      if Actuators_80.F_82_Arm_2_Del
      Status2a_11 = true;
      else
      Status2a_11 = false;
      end
    state ArmCloseDelivery2
      entry:
      Status2a_12 = false;
      during:
      Sensors_70.O_70_SStation;
      if Sensors_70.O_70_SStation
      Status2a_12 = true;
      else
      Status2a_12 = false;
      end
    state ArmArrives_DeliversPart
      entry:
      Status2a_13 = false;
      during:
      Actuators_80.F_82_Suction_On;
      Actuators_80.F_82_Suction_Off;
      Actuators_80.F_82_Arm_2_Del;
      if ~Actuators_80.F_82_Suction_On && ...
      Actuators_80.F_82_Suction_Off && ...
      ~Actuators_80.F_82_Arm_2_Del
      Status2a_13 = true;
      else
      Status2a_13 = false;
      end
    state ArmToMagazine1
      entry:
      Status2a_14 = false;
      during:
      Actuators_80.F_82_Suction_Off;
      Actuators_80.F_82_Arm_2_Mag;
      Actuators_80.F_83_Led_Extra1;
      Control_80.C_85_Part_Del;
      if ~Actuators_80.F_82_Suction_Off && ...
      Actuators_80.F_82_Arm_2_Mag && ...
      Actuators_80.F_83_Led_Extra1 && ...
      Control_80.C_85_Part_Del
      Status2a_14 = true;
      else
      Status2a_14 = false;
      end
    state ArmCloseDeliver3
      entry:
      Status2a_15 = false;
      during:
      Sensors_70.O_70_SStation;
      if Sensors_70.O_70_SStation
      Status2a_15 = true;
      else
      Status2a_15 = false;
      end
    state ArmArrives_Finish
      entry:
      Status2a_16 = false;
      during:
      Actuators_80.F_82_Arm_2_Mag;
      if ~Actuators_80.F_82_Arm_2_Mag;
      Status2a_16 = true;
      else
      Status2a_16 = false;
      end
    state InitialCondition
      entry:
      Status2a_1 = false;
      during:
      Control_80.C_85_Initialization;
      Control_80.C_86_Mag_Parts;
      Control_80.C_82_Profibus;
      Control_80.C_85_Single;
      Sensors_80.O_80_Arm_Mag;
      Sensors_80.O_81_Key_Pos;
      if Control_80.C_85_Initialization&& ...
      Control_80.C_86_Mag_Parts ~= 0 && ...
      Control_80.C_82_Profibus && ...
      Control_80.C_85_Single && ...
      Sensors_80.O_80_Arm_Mag && ...
      Sensors_80.O_81_Key_Pos
      Status2a_1 = true;
      else
      Status2a_1 = false;
      end
    state ArmToDelivery
      entry:
      Status2a_2 = false;
      during:
      Actuators_80.F_82_Arm_2_Del;
      if Actuators_80.F_82_Arm_2_Del
      Status2a_2 = true;
      else
      Status2a_2 = false;
      end
    state ArmCloseDelivery
      entry:
      Status2a_3 = false;
      during:
      Sensors_70.O_70_SStation;
      if Sensors_70.O_70_SStation
      Status2a_3 = true;
      else
      Status2a_3 = false;
      end
    state ArmArrives_FeedsPart
      entry:
      Status2a_4 = false;
      during:
      Actuators_80.F_82_Pist_Adv;
      Actuators_80.F_82_Arm_2_Del;
      if Actuators_80.F_82_Pist_Adv && ...
      ~Actuators_80.F_82_Arm_2_Del
      Status2a_4 = true;
      else
      Status2a_4 = false;
      end
    state PistonStartsMoveForward
      entry:
      Status2a_5 = false;
      during:
      Sensors_80.O_80_Pist_Bck;
      if ~Sensors_80.O_80_Pist_Bck
      Status2a_5 = true;
      else
      Status2a_5 = false;
      end
    state T1
      during:
      Control_80.C_85_Part_Del
      Actuators_80.F_83_Led_Extra1
    (default) -> Distribution_Single.InitialCondition
    Distribution_Single.ArmToMagazine1 -> (junction 650)
    (junction 650) -> Distribution_Single.ArmCloseDeliver3 [order 1] : [Sensors_80.O_80_Arm_Del == false &&...
        |  Status2a_14 == true]
    Distribution_Single.ArmToDelivery -> Distribution_Single.ArmCloseDelivery : [Sensors_80.O_80_Arm_Mag == false &&...
        |  Status2a_2 == true]
    Distribution_Single.ArmCloseDelivery -> Distribution_Single.ArmArrives_FeedsPart : [Sensors_80.O_80_Arm_Del == true && ...
        | Status2a_3 == true]
    Distribution_Single.ArmArrives_DeliversPart -> Distribution_Single.ArmToMagazine1 : [Sensors_80.O_80_Part_Stuck == false && ...
        | Status2a_13 == true]
    Distribution_Single.ArmCloseDelivery2 -> Distribution_Single.ArmArrives_DeliversPart : [Sensors_80.O_80_Arm_Del == true && ...
        | Status2a_12 == true]
    Distribution_Single.ArmArrives_FeedsPart -> Distribution_Single.PistonStartsMoveForward : [Status2a_4 == true]
    Distribution_Single.PistonStartsMoveBackward -> Distribution_Single.ArmToMagazine : [Sensors_80.O_80_Pist_Bck == true && ...
        | Status2a_7 == true]
    Distribution_Single.ArmCloseDeliver1 -> Distribution_Single.ArmArrives_PicksPart : [Sensors_80.O_80_Arm_Mag == true && ...
        | Status2a_9 == true]
    Distribution_Single.PartFed -> Distribution_Single.PistonStartsMoveBackward : [Status2a_6 == true]
    Distribution_Single.ArmToMagazine -> Distribution_Single.ArmCloseDeliver1 : [Sensors_80.O_80_Arm_Del == false &&...
        | Status2a_8 == true]
    Distribution_Single.InitialCondition -> Distribution_Single.ArmToDelivery : [Sensors_80.O_81_Start == true | ...
        | Control_80.C_85_Start == true | ...
        | Control_70.C_75_RQ_Wrong == true | ...
        | (AS_i_70.A_74_CRoute_In80 == true && Sensors_80.O_81_Key_Pos == true) ]
    Distribution_Single.ArmCloseDeliver3 -> Distribution_Single.ArmArrives_Finish : [Sensors_80.O_80_Arm_Mag == true && ...
        | Status2a_15 == true]
    Distribution_Single.ArmToDelivery1 -> Distribution_Single.ArmCloseDelivery2 : [Sensors_80.O_80_Arm_Mag == false &&...
        | Status2a_11 == true]
    Distribution_Single.PistonStartsMoveForward -> Distribution_Single.PartFed : [Sensors_80.O_80_Pist_Fwd == true && ...
        | Status2a_5 == true]
    Distribution_Single.ArmArrives_PicksPart -> Distribution_Single.ArmToDelivery1 : [Sensors_80.O_80_Part_Stuck == true && ...
        | Status2a_10 == true]
    (junction 650) -> (junction 1222) [order 2] : after(4,sec)
    (junction 1222) -> Distribution_Single.T1
  state RBS Output
    state ArmToMagazine1
      entry:
      Status2c_14 = false;
      during:
      Actuators_80.F_82_Suction_Off;
      Actuators_80.F_82_Arm_2_Mag;
      Actuators_80.F_83_Led_Extra1;
      Control_80.C_85_Part_Del;
      if ~Actuators_80.F_82_Suction_Off && ...
      Actuators_80.F_82_Arm_2_Mag && ...
      Actuators_80.F_83_Led_Extra1 && ...
      Control_80.C_85_Part_Del
      Status2c_14 = true;
      else
      Status2c_14 = false;
      end
    state ArmCloseDeliver3
      entry:
      Status2c_15 = false;
      during:
      Sensors_70.O_70_SStation;
      if Sensors_70.O_70_SStation
      Status2c_15 = true;
      else
      Status2c_15 = false;
      end
    state ArmArrives_Finish
      entry:
      Status2c_16 = false;
      during:
      Actuators_80.F_82_Arm_2_Mag;
      if ~Actuators_80.F_82_Arm_2_Mag;
      Status2c_16 = true;
      else
      Status2c_16 = false;
      end
    state ArmToMagazine
      entry:
      Status2c_8 = false;
      during:
      Actuators_80.F_82_Arm_2_Mag;
      if Actuators_80.F_82_Arm_2_Mag
      Status2c_8 = true;
      else
      Status2c_8 = false;
      end
    state ArmCloseDeliver1
      entry:
      Status2c_9 = false;
      during:
      Sensors_70.O_70_SStation;
      if Sensors_70.O_70_SStation
      Status2c_9 = true;
      else
      Status2c_9 = false;
      end
    state ArmArrives_PicksPart
      entry:
      Status2c_10 = false;
      during:
      Actuators_80.F_82_Suction_On;
      Actuators_80.F_82_Arm_2_Mag;
      if Actuators_80.F_82_Suction_On && ...
      ~Actuators_80.F_82_Arm_2_Mag
      Status2c_10 = true;
      else
      Status2c_10 = false;
      end
    state ArmToDelivery1
      entry:
      Status2c_11 = false;
      during:
      Actuators_80.F_82_Arm_2_Del
      if Actuators_80.F_82_Arm_2_Del
      Status2c_11 = true;
      else
      Status2c_11 = false;
      end
    state ArmCloseDelivery2
      entry:
      Status2c_12 = false;
      during:
      Sensors_70.O_70_SStation;
      if Sensors_70.O_70_SStation
      Status2c_12 = true;
      else
      Status2c_12 = false;
      end
    state ArmArrives_DeliversPart
      entry:
      Status2c_13 = false;
      during:
      Actuators_80.F_82_Suction_On;
      Actuators_80.F_82_Suction_Off;
      Actuators_80.F_82_Arm_2_Del;
      if ~Actuators_80.F_82_Suction_On && ...
      Actuators_80.F_82_Suction_Off && ...
      ~Actuators_80.F_82_Arm_2_Del
      Status2c_13 = true;
      else
      Status2c_13 = false;
      end
    state PartDel_CheckLoop
      entry:
      LoopDistCont = false;
      during:
      Control_80.C_85_Part_Del
      Control_80.C_87_RQ_MParts
      if Control_80.C_85_Part_Del && ...
      Control_80.C_87_RQ_MParts == 0
      LoopDistCont = true;
      else
      LoopDistCont = false;
      end
    state InitialCondition
      entry:
      Status2c_1 = false;
      during:
      Control_80.C_85_Initialization;
      Control_80.C_86_Mag_Parts;
      Control_80.C_82_Profibus;
      Control_80.C_85_Continuous;
      Sensors_80.O_80_Arm_Mag;
      Sensors_80.O_81_Key_Pos;
      if Control_80.C_85_Initialization&& ...
      Control_80.C_86_Mag_Parts ~= 0 && ...
      Control_80.C_82_Profibus && ...
      Control_80.C_85_Continuous && ...
      Sensors_80.O_80_Arm_Mag && ...
      Sensors_80.O_81_Key_Pos
      Status2c_1 = true;
      else
      Status2c_1 = false;
      end
    state ArmToDelivery
      entry:
      Status2c_2 = false;
      during:
      Actuators_80.F_82_Arm_2_Del
      if Actuators_80.F_82_Arm_2_Del
      Status2c_2 = true;
      else
      Status2c_2 = false;
      end
    state ArmCloseDelivery
      entry:
      Status2c_3 = false;
      during:
      Sensors_70.O_70_SStation;
      if Sensors_70.O_70_SStation
      Status2c_3 = true;
      else
      Status2c_3 = false;
      end
    state ArmArrives_FeedsPart
      entry:
      Status2b_4 = false;
      during:
      Actuators_80.F_82_Pist_Adv;
      Actuators_80.F_82_Arm_2_Del;
      if Actuators_80.F_82_Pist_Adv && ...
      ~Actuators_80.F_82_Arm_2_Del
      Status2b_4 = true;
      else
      Status2b_4 = false;
      end
    state PistonStartsMoveForward
      entry:
      Status2c_5 = false;
      during:
      Sensors_80.O_80_Pist_Bck;
      if ~Sensors_80.O_80_Pist_Bck
      Status2c_5 = true;
      else
      Status2c_5 = false;
      end
    state PartFed
      entry:
      Status2c_6 = false;
      during:
      Actuators_80.F_82_Pist_Adv;
      if ~Actuators_80.F_82_Pist_Adv
      Status2c_6 = true;
      else
      Status2c_6 = false;
      end
    state PistonStartsMoveBackward
      entry:
      Status2c_7 = false;
      during:
      Sensors_80.O_80_Pist_Fwd;
      if ~Sensors_80.O_80_Pist_Fwd
      Status2c_7 = true;
      else
      Status2c_7 = false;
      end
    state T1
      during:
      Control_80.C_85_Part_Del
      Actuators_80.F_83_Led_Extra1
    RBS.InitialCondition -> RBS.ArmToDelivery : [Sensors_80.O_81_Start == true | ...
        | Control_80.C_85_Start == true | ...
        | Control_70.C_75_RQ_Wrong == true | ...
        | (AS_i_70.A_74_CRoute_In80 == true && Sensors_80.O_81_Key_Pos == true) ]
    RBS.ArmArrives_FeedsPart -> RBS.PistonStartsMoveForward : [Status2b_4 == true]
    RBS.PartDel_CheckLoop -> RBS.ArmToMagazine1 [order 2] : [LoopDistCont == false]
    RBS.ArmCloseDeliver3 -> RBS.ArmArrives_Finish : [Sensors_80.O_80_Arm_Mag == true && ...
        | Status2c_15 == true]
    RBS.ArmCloseDelivery2 -> RBS.ArmArrives_DeliversPart : [Sensors_80.O_80_Arm_Del == true && ...
        | Status2c_12 == true]
    RBS.ArmCloseDelivery -> RBS.ArmArrives_FeedsPart : [Sensors_80.O_80_Arm_Del == true && ...
        | Status2c_3 == true]
    RBS.PistonStartsMoveForward -> RBS.PartFed : [Sensors_80.O_80_Pist_Fwd == true && ...
        | Status2c_5 == true]
    RBS.ArmArrives_DeliversPart -> RBS.PartDel_CheckLoop : [Sensors_80.O_80_Part_Stuck == false && ...
        | Status2c_13 == true]
    RBS.ArmToMagazine1 -> RBS.ArmCloseDeliver3 : [Sensors_80.O_80_Arm_Del == false &&...
        | Status2c_14 == true]
    RBS.ArmArrives_PicksPart -> RBS.ArmToDelivery1 : [Sensors_80.O_80_Part_Stuck == true && ...
        | Status2c_10 == true]
    RBS.PistonStartsMoveBackward -> RBS.ArmToMagazine : [Sensors_80.O_80_Pist_Bck == true && ...
        | Status2c_7 == true]
    RBS.ArmToDelivery -> RBS.ArmCloseDelivery : [Sensors_80.O_80_Arm_Mag == false &&...
        | Status2c_2 == true]
    RBS.ArmToMagazine -> RBS.ArmCloseDeliver1 : [Sensors_80.O_80_Arm_Del == false &&...
        | Status2c_8 == true]
    RBS.ArmCloseDeliver1 -> RBS.ArmArrives_PicksPart : [Sensors_80.O_80_Arm_Mag == true && ...
        | Status2c_9 == true]
    RBS.PartFed -> RBS.PistonStartsMoveBackward : [Status2c_6 == true]
    (default) -> RBS.InitialCondition
    RBS.ArmToDelivery1 -> RBS.ArmCloseDelivery2 : [Sensors_80.O_80_Arm_Mag == false &&...
        | Status2c_11 == true]
    (junction 2192) -> RBS.ArmArrives_FeedsPart
    (junction 2172) -> (junction 2192)
    RBS.PartDel_CheckLoop -> (junction 2182) [order 1] : [LoopDistCont == true]
    RBS.PartDel_CheckLoop -> RBS.T1 [order 3] : after(4,sec)
    (junction 2182) -> (junction 2172)
  note: Handling 1 [50]
  state Distribution_Continuous
    state InitialCondition
      entry:
      Status2b_1 = false;
      during:
      Control_80.C_85_Initialization;
      Control_80.C_86_Mag_Parts;
      Control_80.C_82_Profibus;
      Control_80.C_85_Continuous;
      Sensors_80.O_80_Arm_Mag;
      Sensors_80.O_81_Key_Pos;
      if Control_80.C_85_Initialization&& ...
      Control_80.C_86_Mag_Parts ~= 0 && ...
      Control_80.C_82_Profibus && ...
      Control_80.C_85_Continuous && ...
      Sensors_80.O_80_Arm_Mag && ...
      Sensors_80.O_81_Key_Pos
      Status2a_1 = true;
      else
      Status2b_1 = false;
      end
    state ArmToDelivery
      entry:
      Status2b_2 = false;
      during:
      Actuators_80.F_82_Arm_2_Del
      if Actuators_80.F_82_Arm_2_Del
      Status2b_2 = true;
      else
      Status2b_2 = false;
      end
    state ArmCloseDelivery
      entry:
      Status2b_3 = false;
      during:
      Sensors_70.O_70_SStation;
      if Sensors_70.O_70_SStation
      Status2b_3 = true;
      else
      Status2b_3 = false;
      end
    state ArmArrives_FeedsPart
      entry:
      Status2b_4 = false;
      during:
      Actuators_80.F_82_Pist_Adv;
      Actuators_80.F_82_Arm_2_Del;
      if Actuators_80.F_82_Pist_Adv && ...
      ~Actuators_80.F_82_Arm_2_Del
      Status2b_4 = true;
      else
      Status2b_4 = false;
      end
    state PistonStartsMoveForward
      entry:
      Status2b_5 = false;
      during:
      Sensors_80.O_80_Pist_Bck;
      if ~Sensors_80.O_80_Pist_Bck
      Status2b_5 = true;
      else
      Status2b_5 = false;
      end
    state PartFed
      entry:
      Status2b_6 = false;
      during:
      Actuators_80.F_82_Pist_Adv;
      if ~Actuators_80.F_82_Pist_Adv
      Status2b_6 = true;
      else
      Status2b_6 = false;
      end
    state PistonStartsMoveBackward
      entry:
      Status2b_7 = false;
      during:
      Sensors_80.O_80_Pist_Fwd;
      if ~Sensors_80.O_80_Pist_Fwd
      Status2b_7 = true;
      else
      Status2b_7 = false;
      end
    state ArmToMagazine
      entry:
      Status2b_8 = false;
      during:
      Actuators_80.F_82_Arm_2_Mag;
      if Actuators_80.F_82_Arm_2_Mag
      Status2b_8 = true;
      else
      Status2b_8 = false;
      end
    state ArmCloseDeliver1
      entry:
      Status2b_9 = false;
      during:
      Sensors_70.O_70_SStation;
      if Sensors_70.O_70_SStation
      Status2b_9 = true;
      else
      Status2b_9 = false;
      end
    state ArmArrives_PicksPart
      entry:
      Status2b_10 = false;
      during:
      Actuators_80.F_82_Suction_On;
      Actuators_80.F_82_Arm_2_Mag;
      if Actuators_80.F_82_Suction_On && ...
      ~Actuators_80.F_82_Arm_2_Mag
      Status2b_10 = true;
      else
      Status2b_10 = false;
      end
    state ArmToDelivery1
      entry:
      Status2b_11 = false;
      during:
      Actuators_80.F_82_Arm_2_Del
      if Actuators_80.F_82_Arm_2_Del
      Status2b_11 = true;
      else
      Status2b_11 = false;
      end
    state ArmCloseDelivery2
      entry:
      Status2b_12 = false;
      during:
      Sensors_70.O_70_SStation;
      if Sensors_70.O_70_SStation
      Status2b_12 = true;
      else
      Status2b_12 = false;
      end
    state ArmArrives_DeliversPart
      entry:
      Status2b_13 = false;
      during:
      Actuators_80.F_82_Suction_On;
      Actuators_80.F_82_Suction_Off;
      Actuators_80.F_82_Arm_2_Del;
      if ~Actuators_80.F_82_Suction_On && ...
      Actuators_80.F_82_Suction_Off && ...
      ~Actuators_80.F_82_Arm_2_Del
      Status2b_13 = true;
      else
      Status2b_13 = false;
      end
    state PartDel_CheckLoop
      entry:
      LoopDistCont = false;
      during:
      Control_80.C_85_Part_Del
      Control_80.C_86_Mag_Parts
      if Control_80.C_85_Part_Del && ...
      Control_80.C_86_Mag_Parts ~= 0
      LoopDistCont = true;
      else
      LoopDistCont = false;
      end
    state ArmToMagazine1
      entry:
      Status2b_14 = false;
      during:
      Actuators_80.F_82_Suction_Off;
      Actuators_80.F_82_Arm_2_Mag;
      Actuators_80.F_83_Led_Extra1;
      Control_80.C_85_Part_Del;
      if ~Actuators_80.F_82_Suction_Off && ...
      Actuators_80.F_82_Arm_2_Mag && ...
      Actuators_80.F_83_Led_Extra1 && ...
      Control_80.C_85_Part_Del
      Status2b_14 = true;
      else
      Status2b_14 = false;
      end
    state ArmCloseDeliver3
      entry:
      Status2b_15 = false;
      during:
      Sensors_70.O_70_SStation;
      if Sensors_70.O_70_SStation
      Status2b_15 = true;
      else
      Status2b_15 = false;
      end
    state ArmArrives_Finish
      entry:
      Status2b_16 = false;
      during:
      Actuators_80.F_82_Arm_2_Mag;
      if ~Actuators_80.F_82_Arm_2_Mag;
      Status2b_16 = true;
      else
      Status2b_16 = false;
      end
    state T1
      during:
      Control_80.C_85_Part_Del
      Actuators_80.F_83_Led_Extra1
    Distribution_Continuous.ArmArrives_PicksPart -> Distribution_Continuous.ArmToDelivery1 : [Sensors_80.O_80_Part_Stuck == true && ...
        | Status2b_10 == true]
    Distribution_Continuous.ArmArrives_DeliversPart -> Distribution_Continuous.PartDel_CheckLoop : [Sensors_80.O_80_Part_Stuck == false && ...
        | Status2b_13 == true]
    Distribution_Continuous.ArmCloseDelivery -> Distribution_Continuous.ArmArrives_FeedsPart : [Sensors_80.O_80_Arm_Del == true && ...
        | Status2b_3 == true]
    Distribution_Continuous.ArmArrives_FeedsPart -> Distribution_Continuous.PistonStartsMoveForward : [Status2b_4 == true]
    (default) -> Distribution_Continuous.InitialCondition
    Distribution_Continuous.PartFed -> Distribution_Continuous.PistonStartsMoveBackward : [Status2b_6 == true]
    Distribution_Continuous.PistonStartsMoveForward -> Distribution_Continuous.PartFed : [Sensors_80.O_80_Pist_Fwd == true && ...
        | Status2b_5 == true]
    Distribution_Continuous.ArmToDelivery -> Distribution_Continuous.ArmCloseDelivery : [Sensors_80.O_80_Arm_Mag == false &&...
        | Status2a_2 == true]
    Distribution_Continuous.PistonStartsMoveBackward -> Distribution_Continuous.ArmToMagazine : [Sensors_80.O_80_Pist_Bck == true && ...
        | Status2b_7 == true]
    Distribution_Continuous.ArmCloseDelivery2 -> Distribution_Continuous.ArmArrives_DeliversPart : [Sensors_80.O_80_Arm_Del == true && ...
        | Status2b_12 == true]
    Distribution_Continuous.ArmToMagazine -> Distribution_Continuous.ArmCloseDeliver1 : [Sensors_80.O_80_Arm_Del == false &&...
        |  Status2b_8 == true]
    Distribution_Continuous.ArmCloseDeliver1 -> Distribution_Continuous.ArmArrives_PicksPart : [Sensors_80.O_80_Arm_Mag == true && ...
        | Status2b_9 == true]
    Distribution_Continuous.ArmToDelivery1 -> Distribution_Continuous.ArmCloseDelivery2 : [Sensors_80.O_80_Arm_Mag == false &&...
        |  Status2b_11 == true]
    Distribution_Continuous.InitialCondition -> Distribution_Continuous.ArmToDelivery : [Sensors_80.O_81_Start == true | ...
        | Control_80.C_85_Start == true | ...
        | Control_70.C_75_RQ_Wrong == true | ...
        | (AS_i_70.A_74_CRoute_In80 == true && Sensors_80.O_81_Key_Pos == true) ]
    Distribution_Continuous.ArmToMagazine1 -> Distribution_Continuous.ArmCloseDeliver3 : [Sensors_80.O_80_Arm_Del == false &&...
        | Status2b_14 == true]
    Distribution_Continuous.ArmCloseDeliver3 -> Distribution_Continuous.ArmArrives_Finish : [Sensors_80.O_80_Arm_Mag == true && ...
        | Status2b_15 == true]
    Distribution_Continuous.PartDel_CheckLoop -> Distribution_Continuous.ArmToMagazine1 [order 2] : [LoopDistCont == false]
    (junction 708) -> Distribution_Continuous.ArmArrives_FeedsPart
    (junction 706) -> (junction 708)
    Distribution_Continuous.PartDel_CheckLoop -> (junction 707) [order 1] : [LoopDistCont == true]
    Distribution_Continuous.PartDel_CheckLoop -> Distribution_Continuous.T1 [order 3] : after(4,sec)
    (junction 707) -> (junction 706)
  state PartToProcessing2
    state FinishesProcess
      entry:
      Status5_13 = false;
      during:
      Control_90.C_95_PD_Proc;
      if Control_90.C_95_PD_Proc
      Status5_13 = true;
      else
      Status5_13 = false;
      end
    state ClawBeginsAscend
      entry:
      Status5_12 = false;
      during:
      Sensors_90.O_90_Part_in_Claw;
      if ~Sensors_90.O_90_Part_in_Claw
      Status5_12 = true;
      else
      Status5_12 = false;
      end
    state DeliversPart
      entry:
      Status5_11 = false;
      during:
      Actuators_90.F_92_Claw_Down;
      Actuators_90.F_92_Close_Claw;
      if ~Actuators_90.F_92_Claw_Down && ...
      ~Actuators_90.F_92_Close_Claw
      Status5_11 = true;
      else
      Status5_11 = false;
      end
    state ClawDescent
      entry:
      Status5_10 = false;
      during:
      Sensors_90.O_90_Claw_Low;
      Sensors_90.O_90_Claw_High;
      if Sensors_90.O_90_Claw_Low && ...
      ~Sensors_90.O_90_Claw_High
      Status5_10 = true;
      else
      Status5_10 = false;
      end
    state ArmArrives
      entry:
      Status5_9 = false;
      during:
      Actuators_90.F_92_Claw_2_Del;
      Actuators_90.F_92_Claw_Down;
      if ~Actuators_90.F_92_Claw_2_Del && ...
      Actuators_90.F_92_Claw_Down
      Status5_9 = true;
      else
      Status5_9 = false;
      end
    state ArmPassesStorage
      entry:
      Status5_8 = false;
      during:
      Sensors_90.O_90_Claw_Reserve
      if ~Sensors_90.O_90_Claw_Reserve
      Status5_8 = true;
      else
      Status5_8 = false;
      end
    state ArmStartsMovement
      entry:
      Status5_7 = false;
      during:
      Sensors_90.O_90_Claw_Reserve
      if Sensors_90.O_90_Claw_Reserve
      Status5_7 = true;
      else
      Status5_7 = false;
      end
    state ClawFinishesAscend
      entry:
      Status5_6 = false;
      during:
      Actuators_90.F_92_Claw_2_Del;
      if Actuators_90.F_92_Claw_2_Del
      Status5_6 = true;
      else
      Status5_6 = false;
      end
    state PartLeavesCart
      entry:
      Status5_5 = false;
      during:
      AS_i_90.A_94_Cart_Full;
      if ~AS_i_90.A_94_Cart_Full
      Status5_5 = true;
      else
      Status5_5 = false;
      end
    state PartPickup_BeginsAscend
      entry:
      Status5_4 = false;
      during:
      Actuators_90.F_92_Claw_Down;
      Sensors_90.O_90_Claw_Low;
      if ~Actuators_90.F_92_Claw_Down && ...
      ~Sensors_90.O_90_Claw_Low
      Status5_4 = true;
      else
      Status5_4 = false;
      end
    state ClawFinishesDescent
      entry:
      Status5_3 = false;
      during:
      Actuators_90.F_92_Close_Claw;
      if Actuators_90.F_92_Close_Claw
      Status5_3 = true;
      else
      Status5_3 = false;
      end
    state ClawBeginsDescent
      entry:
      Status5_2 = false;
      during:
      Actuators_90.F_92_Claw_Down;
      Control_90.C_95_PD_Proc;
      Control_90.C_95_PD_Cart;
      Sensors_90.O_90_Claw_High;
      if Actuators_90.F_92_Claw_Down && ...
      ~Control_90.C_95_PD_Proc && ...
      ~Control_90.C_95_PD_Cart && ...
      ~Sensors_90.O_90_Claw_High
      Status5_2 = true;
      else
      Status5_2 = false;
      end
    state InitialCondition
      entry:
      Status5_1 = false;
      during:
      AS_i_90.A_94_Cart_Full;
      Control_90.C_95_Initialization;
      Control_90.C_95_Cart2Del;
      Control_90.C_92_Profibus;
      Sensors_90.O_91_Key_Pos;
      if AS_i_90.A_94_Cart_Full && ...
      Control_90.C_95_Initialization && ...
      Control_90.C_95_Cart2Del && ...
      Control_90.C_92_Profibus && ...
      Sensors_90.O_91_Key_Pos
      Status5_1 = true;
      else
      Status5_1 = false;
      end
    (default) -> PartToProcessing2.InitialCondition
    PartToProcessing2.ArmStartsMovement -> PartToProcessing2.ArmPassesStorage : [Sensors_90.O_90_Claw_Reserve == false && ...
        | Status5_7 == true]
    PartToProcessing2.ClawBeginsAscend -> PartToProcessing2.FinishesProcess : [Sensors_90.O_90_Claw_High == true && ...
        | Status5_12 == true]
    PartToProcessing2.DeliversPart -> PartToProcessing2.ClawBeginsAscend : [Sensors_90.O_90_Claw_Low && ...
        | Status5_11 == true]
    PartToProcessing2.ArmArrives -> PartToProcessing2.ClawDescent : [Sensors_90.O_90_Claw_High == false && ...
        | Status5_9 == true]
    PartToProcessing2.ClawFinishesAscend -> PartToProcessing2.ArmStartsMovement : [Sensors_90.O_90_Claw_Cart == false && ...
        | Status5_6 == true]
    PartToProcessing2.ClawFinishesDescent -> PartToProcessing2.PartPickup_BeginsAscend : [Sensors_90.O_90_Part_in_Claw == true && ...
        | Status5_3 == true]
    PartToProcessing2.PartLeavesCart -> PartToProcessing2.ClawFinishesAscend : [Sensors_90.O_90_Claw_High == true && ...
        | Status5_5 == true]
    PartToProcessing2.PartPickup_BeginsAscend -> PartToProcessing2.PartLeavesCart : [AS_i_90.A_94_Optic == false && ...
        | Status5_4 == true]
    PartToProcessing2.ClawDescent -> PartToProcessing2.DeliversPart : [Sensors_100.O_100_PInit_Pos == true && ...
        | Status5_10 == true]
    PartToProcessing2.ClawBeginsDescent -> PartToProcessing2.ClawFinishesDescent : [Sensors_90.O_90_Claw_Low == true && ...
        | Status5_2 == true]
    PartToProcessing2.InitialCondition -> PartToProcessing2.ClawBeginsDescent : [AS_i_90.A_94_CRoute_In == true && ...
        |  Status5_1 == true]
    PartToProcessing2.ArmPassesStorage -> PartToProcessing2.ArmArrives : [Sensors_90.O_90_Claw_Del == true && ...
        | Status5_8 == true]
  state Requested_Delivery
    state Part_HeightSensor
      entry:
      Status3b_8 = false;
      during:
      Actuators_70.F_72_Eject_Part;
      Sensors_70.O_70_Pist_Bck;
      Sensors_70.O_70_SPart_Height
      if Actuators_70.F_72_Eject_Part && ...
      ~Sensors_70.O_70_Pist_Bck && ...
      ~Sensors_70.O_70_SPart_Height
      Status3b_8 = true
      else
      Status3b_8 = false
      end
    state Piston_Back
      entry:
      Status3b_10 = false;
      during:
      Actuators_70.F_72_Eject_Part
      if ~Actuators_70.F_72_Eject_Part
      Status3b_10 = true
      else
      Status3b_10 = false
      end
    state Elevator_StartsMovingDown
      entry:
      Status3b_11 = false;
      during:
      Actuators_70.F_72_Elev_Down;
      Actuators_70.F_72_Elev_Up;
      if Actuators_70.F_72_Elev_Down && ...
      ~Actuators_70.F_72_Elev_Up
      Status3b_11 = true
      else
      Status3b_11 = false
      end
    state Elevator_MiddleDown
      entry:
      Status3b_12 = false;
      during:
      Sensors_70.O_70_SStation;
      if ~Sensors_70.O_70_SStation
      Status3b_12 = true
      else
      Status3b_12 = false
      end
    state Elevator_InductiveDown
      entry:
      Status3b_13 = false;
      during:
      Sensors_70.O_70_SInductive;
      if ~Sensors_70.O_70_SInductive
      Status3b_13 = true
      else
      Status3b_13 = false
      end
    state InitialCondition
      entry:
      Status3b_1 = false;
      during:
      AS_i_70.A_74_Cart_Full;
      Control_70.C_75_Initialization;
      Control_70.C_72_Profibus;
      Control_70.C_75_Requested;
      Sensors_70.O_70_SPart;
      Sensors_70.O_71_Key_Pos;
      if ~AS_i_70.A_74_Cart_Full && ...
      Control_70.C_75_Initialization && ...
      Control_70.C_72_Profibus && ...
      Control_70.C_75_Requested && ...
      ~Sensors_70.O_70_SPart && ...
      Sensors_70.O_71_Key_Pos
      Status3b_1 = true;
      else
      Status3b_1 = false;
      end
    state Part_Arrives
      entry:
      Status3b_2 = false;
      during:
      Control_70.C_75_ID_Delivery2;
      Sensors_70.O_70_SInductive;
      Sensors_70.O_70_SPart;
      Sensors_80.O_80_Arm_Mag;
      if Sensors_70.O_70_SPart && ...
      ((Sensors_70.O_70_SInductive && ...
      Control_70.C_75_ID_Delivery2) | ...
      (~Sensors_70.O_70_SInductive && ...
      ~Control_70.C_75_ID_Delivery2)) && ...
      ~Sensors_80.O_80_Arm_Mag
      Status3b_2 = true;
      else
      Status3b_2 =false;
      end
    state Elevator_Up
      entry:
      Status3b_3 = false;
      during:
      Actuators_70.F_72_Elev_Up;
      if Actuators_70.F_72_Elev_Up
      Status3b_3 = true
      else
      Status3b_3 = false
      end
    state Elevator_StartsMovingUp
      entry:
      Status3b_4 = false;
      during:
      Sensors_70.O_70_SInductive;
      if ~Sensors_70.O_70_SInductive
      Status3b_4 = true
      else
      Status3b_4 = false
      end
    state Elevator_MiddleUp
      entry:
      Status3b_5 = false;
      during:
      Sensors_70.O_70_SStation;
      if ~Sensors_70.O_70_SStation
      Status3b_5 = true
      else
      Status3b_5 = false
      end
    state Elevator_High_Identify_Part
      entry:
      Status3b_6 = false;
      during:
      MetalicPart;
      Control_70.C_75_ID_Delivery1;
      Control_70.C_75_ID_Delivery2;
      Sensors_70.O_70_SPart_Height;
      if MetalicPart && ...
      Control_70.C_75_ID_Delivery2 && ...
      ~Control_70.C_75_ID_Delivery1;
      Status3b_6 = true
      end
      if ~MetalicPart && ...
      Control_70.C_75_ID_Delivery1 && ...
      ((Sensors_70.O_70_SPart_Height && ...
      Control_70.C_75_ID_Delivery2) | ...
      (~Sensors_70.O_70_SPart_Height && ...
      ~Control_70.C_75_ID_Delivery2))
      Status3b_6=true
      end
    state CheckPart
      entry:
      Part_Equal = false;
      Part_Different = false;
      during:
      Control_70.C_75_ID_Delivery1;
      Control_70.C_75_ID_Delivery2;
      Control_70.C_75_RQ_Delivery1;
      Control_70.C_75_RQ_Delivery2;
      if (Control_70.C_75_ID_Delivery1 == ...
      Control_70.C_75_RQ_Delivery1) && ...
      (Control_70.C_75_ID_Delivery2 == ...
      Control_70.C_75_RQ_Delivery2)
      Part_Equal = true
      else
      Part_Different = true
      end
    state Pushes_Part
      entry:
      Status3b_7 = false;
      during:
      Actuators_70.F_72_Eject_Part;
      Actuators_70.F_72_Air_On;
      Sensors_70.O_70_SPart;
      if Actuators_70.F_72_Eject_Part && ...
      Actuators_70.F_72_Air_On && ...
      ~Sensors_70.O_70_SPart
      Status3b_7 = true
      else
      Status3b_7 = false
      end
    state Elevator_Down
      entry:
      Status3b_14 = false;
      during:
      AS_i_70.A_74_CRoute_Out;
      Actuators_70.F_72_Elev_Down;
      Control_70.C_75_Part_Del;
      if AS_i_70.A_74_CRoute_Out && ...
      ~Actuators_70.F_72_Elev_Down&& ...
      Control_70.C_75_Part_Del
      Status3b_14 = true
      else
      Status3b_14 = false
      end
    state Part_ArrivesAtCart
      entry:
      Status3b_9 = false;
      during:
      AS_i_70.A_74_Cart_Full;
      AS_i_70.A_74_Optic;
      Actuators_70.F_72_Air_On;
      Actuators_70.F_73_Led_Extra2
      if AS_i_70.A_74_Optic && ...
      AS_i_70.A_74_Cart_Full && ...
      ~Actuators_70.F_72_Air_On && ...
      Actuators_70.F_73_Led_Extra2;
      Status3b_9 = true
      else
      Status3b_9 = false
      end
    state End_Process
      entry:
      Status3b15 = false;
      during:
      AS_i_70.A_74_CRoute_Out;
      if  ~AS_i_70.A_74_CRoute_Out;
      Status3b_15 = true
      else
      Status3b_15 = false
      end
    state Metalic_Identify
      entry:
      MetalicPart = false;
      during:
      Sensors_70.O_70_SInductive;
      if Sensors_70.O_70_SInductive
      MetalicPart = true
      else
      MetalicPart = false
      end
    state Elevator_StartsMovingDown1
      entry:
      Status3b_16 = false;
      during:
      Actuators_70.F_72_Elev_Down;
      Actuators_70.F_72_Elev_Up;
      if Actuators_70.F_72_Elev_Down && ...
      ~Actuators_70.F_72_Elev_Up
      Status3b_16 = true
      else
      Status3b_16 = false
      end
    state Elevator_MiddleDown1
      entry:
      Status3b_17 = false;
      during:
      Sensors_70.O_70_SStation;
      if ~Sensors_70.O_70_SStation
      Status3b_17 = true
      else
      Status3b_17 = false
      end
    state Elevator_InductiveDown1
      entry:
      Status3b_18 = false;
      during:
      Sensors_70.O_70_SInductive;
      if ~Sensors_70.O_70_SInductive
      Status3b_18 = true
      else
      Status3b_18 = false
      end
    state Elevator_Down1
      entry:
      Status3b_19 = false;
      during:
      Actuators_70.F_72_Eject_Part
      Actuators_70.F_72_Elev_Down
      if Actuators_70.F_72_Eject_Part && ...
      ~Actuators_70.F_72_Elev_Down
      Status3b_19 = true
      else
      Status3b_19 = false
      end
    state Piston_Back1
      entry:
      Status3b_20 = false;
      during:
      Actuators_70.F_72_Eject_Part
      Sensors_70.O_70_Pist_Bck;
      Sensors_70.O_70_SPart
      Control_70.C_75_RQ_Wrong;
      if ~Actuators_70.F_72_Eject_Part && ...
      Sensors_70.O_70_Pist_Bck && ...
      ~Sensors_70.O_70_SPart && ...
      Control_70.C_75_RQ_Wrong;
      Status3b_20 = true
      else
      Status3b_20 = false
      end
    (default) -> Requested_Delivery.InitialCondition
    Requested_Delivery.Elevator_StartsMovingDown -> Requested_Delivery.Elevator_MiddleDown : [Status3b_11 == true && ...
        | Sensors_70.O_70_SStation == true]
    Requested_Delivery.Piston_Back -> Requested_Delivery.Elevator_StartsMovingDown : [Status3b_10 == true && ...
        | Sensors_70.O_70_Pist_Bck == true]
    Requested_Delivery.Elevator_MiddleDown -> Requested_Delivery.Elevator_InductiveDown : [Status3b_12 == true && ...
        | Sensors_70.O_70_SInductive == true]
    Requested_Delivery.Part_Arrives -> Requested_Delivery.Elevator_Up : [Status3b_2 == true && ...
        | Sensors_80.O_80_Arm_Mag == true ]
    Requested_Delivery.Pushes_Part -> Requested_Delivery.Part_HeightSensor : [Status3b_7 == true && ...
        | Sensors_70.O_70_Pist_Bck == false]
    Requested_Delivery.Elevator_Up -> Requested_Delivery.Elevator_StartsMovingUp : [Status3b_3 == true && ...
        | Sensors_70.O_70_SInductive == true ]
    Requested_Delivery.Elevator_StartsMovingUp -> Requested_Delivery.Elevator_MiddleUp : [Status3b_4 == true && ...
        | Sensors_70.O_70_SStation == true]
    Requested_Delivery.Elevator_MiddleUp -> Requested_Delivery.Elevator_High_Identify_Part : [Status3b_5 == true && ...
        | Sensors_70.O_70_Elev_High == true]
    Requested_Delivery.Elevator_InductiveDown -> Requested_Delivery.Elevator_Down : [Status3a_13 == true && ...
        | Sensors_70.O_70_Elev_Low == true]
    Requested_Delivery.Part_HeightSensor -> (junction 1412)
    (junction 1412) -> Requested_Delivery.Piston_Back [order 1] : [Status3b_8 == true && ...
        | after (2,sec)]
    Requested_Delivery.Elevator_High_Identify_Part -> CheckPart : [Status3b_6 == true && ...
        | after (2,sec)]
    CheckPart -> (junction 1378)
    (junction 1378) -> Requested_Delivery.Pushes_Part [order 1] : [Part_Equal == true && ...
        | after (2,sec)]
    Requested_Delivery.InitialCondition -> (junction 1372) : [Status3a_1 == true && ...
        | Sensors_70.O_70_SPart == true]
    (junction 1372) -> Requested_Delivery.Part_Arrives [order 1]
    (junction 1412) -> (junction 1410) [order 2] : [Status3a_8 == true && ...
        | AS_i_70.A_74_Optic == true]
    (junction 1378) -> (junction 952) [order 2] : [Part_Different == true && ...
        | after (2,sec)]
    (junction 1372) -> (junction 1376) [order 2]
    Requested_Delivery.Elevator_Down -> Requested_Delivery.End_Process : after (2,sec)
    (junction 1410) -> Requested_Delivery.Part_ArrivesAtCart
    (junction 1376) -> Requested_Delivery.Metalic_Identify
    Elevator_MiddleDown1 -> Elevator_InductiveDown1 : [Status3b_17 == true && ...
        | Sensors_70.O_70_SInductive == true]
    Elevator_StartsMovingDown1 -> Elevator_MiddleDown1 : [Status3b_16 == true && ...
        | Sensors_70.O_70_SStation == true]
    Elevator_Down1 -> Piston_Back1 : [Status3b_19 == true && ...
        | Sensors_70.O_70_Pist_Bck == false]
    (junction 952) -> Elevator_StartsMovingDown1
    Elevator_InductiveDown1 -> Elevator_Down1 : [Status3b_18 == true && ...
        | Sensors_70.O_70_Elev_Low == true]
  state RSB Output
    state ArmToMagazine1
      entry:
      Status2c_14 = false;
      during:
      Actuators_80.F_82_Suction_Off;
      Actuators_80.F_82_Arm_2_Mag;
      Actuators_80.F_83_Led_Extra1;
      Control_80.C_85_Part_Del;
      if ~Actuators_80.F_82_Suction_Off && ...
      Actuators_80.F_82_Arm_2_Mag && ...
      Actuators_80.F_83_Led_Extra1 && ...
      Control_80.C_85_Part_Del
      Status2c_14 = true;
      else
      Status2c_14 = false;
      end
    state ArmCloseDeliver3
      entry:
      Status2c_15 = false;
      during:
      Sensors_70.O_70_SStation;
      if Sensors_70.O_70_SStation
      Status2c_15 = true;
      else
      Status2c_15 = false;
      end
    state ArmArrives_Finish
      entry:
      Status2c_16 = false;
      during:
      Actuators_80.F_82_Arm_2_Mag;
      if ~Actuators_80.F_82_Arm_2_Mag;
      Status2c_16 = true;
      else
      Status2c_16 = false;
      end
    state ArmToMagazine
      entry:
      Status2c_8 = false;
      during:
      Actuators_80.F_82_Arm_2_Mag;
      if Actuators_80.F_82_Arm_2_Mag
      Status2c_8 = true;
      else
      Status2c_8 = false;
      end
    state ArmCloseDeliver1
      entry:
      Status2c_9 = false;
      during:
      Sensors_70.O_70_SStation;
      if Sensors_70.O_70_SStation
      Status2c_9 = true;
      else
      Status2c_9 = false;
      end
    state ArmArrives_PicksPart
      entry:
      Status2c_10 = false;
      during:
      Actuators_80.F_82_Suction_On;
      Actuators_80.F_82_Arm_2_Mag;
      if Actuators_80.F_82_Suction_On && ...
      ~Actuators_80.F_82_Arm_2_Mag
      Status2c_10 = true;
      else
      Status2c_10 = false;
      end
    state ArmToDelivery1
      entry:
      Status2c_11 = false;
      during:
      Actuators_80.F_82_Arm_2_Del
      if Actuators_80.F_82_Arm_2_Del
      Status2c_11 = true;
      else
      Status2c_11 = false;
      end
    state ArmCloseDelivery2
      entry:
      Status2c_12 = false;
      during:
      Sensors_70.O_70_SStation;
      if Sensors_70.O_70_SStation
      Status2c_12 = true;
      else
      Status2c_12 = false;
      end
    state ArmArrives_DeliversPart
      entry:
      Status2c_13 = false;
      during:
      Actuators_80.F_82_Suction_On;
      Actuators_80.F_82_Suction_Off;
      Actuators_80.F_82_Arm_2_Del;
      if ~Actuators_80.F_82_Suction_On && ...
      Actuators_80.F_82_Suction_Off && ...
      ~Actuators_80.F_82_Arm_2_Del
      Status2c_13 = true;
      else
      Status2c_13 = false;
      end
    state PartDel_CheckLoop
      entry:
      LoopDistCont = false;
      during:
      Control_80.C_85_Part_Del
      Control_80.C_87_RQ_MParts
      if Control_80.C_85_Part_Del && ...
      Control_80.C_87_RQ_MParts == 0
      LoopDistCont = true;
      else
      LoopDistCont = false;
      end
    state InitialCondition
      entry:
      Status2c_1 = false;
      during:
      Control_80.C_85_Initialization;
      Control_80.C_86_Mag_Parts;
      Control_80.C_82_Profibus;
      Control_80.C_85_Continuous;
      Sensors_80.O_80_Arm_Mag;
      Sensors_80.O_81_Key_Pos;
      if Control_80.C_85_Initialization&& ...
      Control_80.C_86_Mag_Parts ~= 0 && ...
      Control_80.C_82_Profibus && ...
      Control_80.C_85_Continuous && ...
      Sensors_80.O_80_Arm_Mag && ...
      Sensors_80.O_81_Key_Pos
      Status2c_1 = true;
      else
      Status2c_1 = false;
      end
    state ArmToDelivery
      entry:
      Status2c_2 = false;
      during:
      Actuators_80.F_82_Arm_2_Del
      if Actuators_80.F_82_Arm_2_Del
      Status2c_2 = true;
      else
      Status2c_2 = false;
      end
    state ArmCloseDelivery
      entry:
      Status2c_3 = false;
      during:
      Sensors_70.O_70_SStation;
      if Sensors_70.O_70_SStation
      Status2c_3 = true;
      else
      Status2c_3 = false;
      end
    state ArmArrives_FeedsPart
      entry:
      Status2b_4 = false;
      during:
      Actuators_80.F_82_Pist_Adv;
      Actuators_80.F_82_Arm_2_Del;
      if Actuators_80.F_82_Pist_Adv && ...
      ~Actuators_80.F_82_Arm_2_Del
      Status2b_4 = true;
      else
      Status2b_4 = false;
      end
    state PistonStartsMoveForward
      entry:
      Status2c_5 = false;
      during:
      Sensors_80.O_80_Pist_Bck;
      if ~Sensors_80.O_80_Pist_Bck
      Status2c_5 = true;
      else
      Status2c_5 = false;
      end
    state PartFed
      entry:
      Status2c_6 = false;
      during:
      Actuators_80.F_82_Pist_Adv;
      if ~Actuators_80.F_82_Pist_Adv
      Status2c_6 = true;
      else
      Status2c_6 = false;
      end
    state PistonStartsMoveBackward
      entry:
      Status2c_7 = false;
      during:
      Sensors_80.O_80_Pist_Fwd;
      if ~Sensors_80.O_80_Pist_Fwd
      Status2c_7 = true;
      else
      Status2c_7 = false;
      end
    state T1
      during:
      Control_80.C_85_Part_Del
      Actuators_80.F_83_Led_Extra1
    RSB.InitialCondition -> RSB.ArmToDelivery : [Sensors_80.O_81_Start == true | ...
        | Control_80.C_85_Start == true | ...
        | Control_70.C_75_RQ_Wrong == true | ...
        | (AS_i_70.A_74_CRoute_In80 == true && Sensors_80.O_81_Key_Pos == true) ]
    RSB.ArmArrives_FeedsPart -> RSB.PistonStartsMoveForward : [Status2b_4 == true]
    RSB.PartDel_CheckLoop -> RSB.ArmToMagazine1 [order 2] : [LoopDistCont == false]
    RSB.ArmCloseDeliver3 -> RSB.ArmArrives_Finish : [Sensors_80.O_80_Arm_Mag == true && ...
        | Status2c_15 == true]
    RSB.ArmCloseDelivery2 -> RSB.ArmArrives_DeliversPart : [Sensors_80.O_80_Arm_Del == true && ...
        | Status2c_12 == true]
    RSB.ArmCloseDelivery -> RSB.ArmArrives_FeedsPart : [Sensors_80.O_80_Arm_Del == true && ...
        | Status2c_3 == true]
    RSB.PistonStartsMoveForward -> RSB.PartFed : [Sensors_80.O_80_Pist_Fwd == true && ...
        | Status2c_5 == true]
    RSB.ArmArrives_DeliversPart -> RSB.PartDel_CheckLoop : [Sensors_80.O_80_Part_Stuck == false && ...
        | Status2c_13 == true]
    RSB.ArmToMagazine1 -> RSB.ArmCloseDeliver3 : [Sensors_80.O_80_Arm_Del == false &&...
        | Status2c_14 == true]
    RSB.ArmArrives_PicksPart -> RSB.ArmToDelivery1 : [Sensors_80.O_80_Part_Stuck == true && ...
        | Status2c_10 == true]
    RSB.PistonStartsMoveBackward -> RSB.ArmToMagazine : [Sensors_80.O_80_Pist_Bck == true && ...
        | Status2c_7 == true]
    RSB.ArmToDelivery -> RSB.ArmCloseDelivery : [Sensors_80.O_80_Arm_Mag == false &&...
        | Status2c_2 == true]
    RSB.ArmToMagazine -> RSB.ArmCloseDeliver1 : [Sensors_80.O_80_Arm_Del == false &&...
        | Status2c_8 == true]
    RSB.ArmCloseDeliver1 -> RSB.ArmArrives_PicksPart : [Sensors_80.O_80_Arm_Mag == true && ...
        | Status2c_9 == true]
    RSB.PartFed -> RSB.PistonStartsMoveBackward : [Status2c_6 == true]
    (default) -> RSB.InitialCondition
    RSB.ArmToDelivery1 -> RSB.ArmCloseDelivery2 : [Sensors_80.O_80_Arm_Mag == false &&...
        | Status2c_11 == true]
    (junction 2232) -> RSB.ArmArrives_FeedsPart
    (junction 2215) -> (junction 2232)
    RSB.PartDel_CheckLoop -> (junction 2220) [order 1] : [LoopDistCont == true]
    RSB.PartDel_CheckLoop -> RSB.T1 [order 3] : after(4,sec)
    (junction 2220) -> (junction 2215)
  state Distribution_Counted
    state ArmToMagazine1
      entry:
      Status2c_14 = false;
      during:
      Actuators_80.F_82_Suction_Off;
      Actuators_80.F_82_Arm_2_Mag;
      Actuators_80.F_83_Led_Extra1;
      Control_80.C_85_Part_Del;
      if ~Actuators_80.F_82_Suction_Off && ...
      Actuators_80.F_82_Arm_2_Mag && ...
      Actuators_80.F_83_Led_Extra1 && ...
      Control_80.C_85_Part_Del
      Status2c_14 = true;
      else
      Status2c_14 = false;
      end
    state ArmCloseDeliver3
      entry:
      Status2c_15 = false;
      during:
      Sensors_70.O_70_SStation;
      if Sensors_70.O_70_SStation
      Status2c_15 = true;
      else
      Status2c_15 = false;
      end
    state ArmArrives_Finish
      entry:
      Status2c_16 = false;
      during:
      Actuators_80.F_82_Arm_2_Mag;
      if ~Actuators_80.F_82_Arm_2_Mag;
      Status2c_16 = true;
      else
      Status2c_16 = false;
      end
    state ArmToMagazine
      entry:
      Status2c_8 = false;
      during:
      Actuators_80.F_82_Arm_2_Mag;
      if Actuators_80.F_82_Arm_2_Mag
      Status2c_8 = true;
      else
      Status2c_8 = false;
      end
    state ArmCloseDeliver1
      entry:
      Status2c_9 = false;
      during:
      Sensors_70.O_70_SStation;
      if Sensors_70.O_70_SStation
      Status2c_9 = true;
      else
      Status2c_9 = false;
      end
    state ArmArrives_PicksPart
      entry:
      Status2c_10 = false;
      during:
      Actuators_80.F_82_Suction_On;
      Actuators_80.F_82_Arm_2_Mag;
      if Actuators_80.F_82_Suction_On && ...
      ~Actuators_80.F_82_Arm_2_Mag
      Status2c_10 = true;
      else
      Status2c_10 = false;
      end
    state ArmToDelivery1
      entry:
      Status2c_11 = false;
      during:
      Actuators_80.F_82_Arm_2_Del
      if Actuators_80.F_82_Arm_2_Del
      Status2c_11 = true;
      else
      Status2c_11 = false;
      end
    state ArmCloseDelivery2
      entry:
      Status2c_12 = false;
      during:
      Sensors_70.O_70_SStation;
      if Sensors_70.O_70_SStation
      Status2c_12 = true;
      else
      Status2c_12 = false;
      end
    state ArmArrives_DeliversPart
      entry:
      Status2c_13 = false;
      during:
      Actuators_80.F_82_Suction_On;
      Actuators_80.F_82_Suction_Off;
      Actuators_80.F_82_Arm_2_Del;
      if ~Actuators_80.F_82_Suction_On && ...
      Actuators_80.F_82_Suction_Off && ...
      ~Actuators_80.F_82_Arm_2_Del
      Status2c_13 = true;
      else
      Status2c_13 = false;
      end
    state PartDel_CheckLoop
      entry:
      LoopDistCont = false;
      during:
      Control_80.C_85_Part_Del
      Control_80.C_87_RQ_MParts
      if Control_80.C_85_Part_Del && ...
      Control_80.C_87_RQ_MParts == 0
      LoopDistCont = true;
      else
      LoopDistCont = false;
      end
    state InitialCondition
      entry:
      Status2c_1 = false;
      during:
      Control_80.C_85_Initialization;
      Control_80.C_86_Mag_Parts;
      Control_80.C_82_Profibus;
      Control_80.C_85_Continuous;
      Sensors_80.O_80_Arm_Mag;
      Sensors_80.O_81_Key_Pos;
      if Control_80.C_85_Initialization&& ...
      Control_80.C_86_Mag_Parts ~= 0 && ...
      Control_80.C_82_Profibus && ...
      Control_80.C_85_Continuous && ...
      Sensors_80.O_80_Arm_Mag && ...
      Sensors_80.O_81_Key_Pos
      Status2c_1 = true;
      else
      Status2c_1 = false;
      end
    state ArmToDelivery
      entry:
      Status2c_2 = false;
      during:
      Actuators_80.F_82_Arm_2_Del
      if Actuators_80.F_82_Arm_2_Del
      Status2c_2 = true;
      else
      Status2c_2 = false;
      end
    state ArmCloseDelivery
      entry:
      Status2c_3 = false;
      during:
      Sensors_70.O_70_SStation;
      if Sensors_70.O_70_SStation
      Status2c_3 = true;
      else
      Status2c_3 = false;
      end
    state ArmArrives_FeedsPart
      entry:
      Status2b_4 = false;
      during:
      Actuators_80.F_82_Pist_Adv;
      Actuators_80.F_82_Arm_2_Del;
      if Actuators_80.F_82_Pist_Adv && ...
      ~Actuators_80.F_82_Arm_2_Del
      Status2b_4 = true;
      else
      Status2b_4 = false;
      end
    state PistonStartsMoveForward
      entry:
      Status2c_5 = false;
      during:
      Sensors_80.O_80_Pist_Bck;
      if ~Sensors_80.O_80_Pist_Bck
      Status2c_5 = true;
      else
      Status2c_5 = false;
      end
    state PartFed
      entry:
      Status2c_6 = false;
      during:
      Actuators_80.F_82_Pist_Adv;
      if ~Actuators_80.F_82_Pist_Adv
      Status2c_6 = true;
      else
      Status2c_6 = false;
      end
    state PistonStartsMoveBackward
      entry:
      Status2c_7 = false;
      during:
      Sensors_80.O_80_Pist_Fwd;
      if ~Sensors_80.O_80_Pist_Fwd
      Status2c_7 = true;
      else
      Status2c_7 = false;
      end
    state T1
      during:
      Control_80.C_85_Part_Del
      Actuators_80.F_83_Led_Extra1
    Distribution_Counted.InitialCondition -> Distribution_Counted.ArmToDelivery : [Sensors_80.O_81_Start == true | ...
        | Control_80.C_85_Start == true | ...
        | Control_70.C_75_RQ_Wrong == true | ...
        | (AS_i_70.A_74_CRoute_In80 == true && Sensors_80.O_81_Key_Pos == true) ]
    Distribution_Counted.ArmArrives_FeedsPart -> Distribution_Counted.PistonStartsMoveForward : [Status2b_4 == true]
    Distribution_Counted.PartDel_CheckLoop -> Distribution_Counted.ArmToMagazine1 [order 2] : [LoopDistCont == false]
    Distribution_Counted.ArmCloseDeliver3 -> Distribution_Counted.ArmArrives_Finish : [Sensors_80.O_80_Arm_Mag == true && ...
        | Status2c_15 == true]
    Distribution_Counted.ArmCloseDelivery2 -> Distribution_Counted.ArmArrives_DeliversPart : [Sensors_80.O_80_Arm_Del == true && ...
        | Status2c_12 == true]
    Distribution_Counted.ArmCloseDelivery -> Distribution_Counted.ArmArrives_FeedsPart : [Sensors_80.O_80_Arm_Del == true && ...
        | Status2c_3 == true]
    Distribution_Counted.PistonStartsMoveForward -> Distribution_Counted.PartFed : [Sensors_80.O_80_Pist_Fwd == true && ...
        | Status2c_5 == true]
    Distribution_Counted.ArmArrives_DeliversPart -> Distribution_Counted.PartDel_CheckLoop : [Sensors_80.O_80_Part_Stuck == false && ...
        | Status2c_13 == true]
    Distribution_Counted.ArmToMagazine1 -> Distribution_Counted.ArmCloseDeliver3 : [Sensors_80.O_80_Arm_Del == false &&...
        | Status2c_14 == true]
    Distribution_Counted.ArmArrives_PicksPart -> Distribution_Counted.ArmToDelivery1 : [Sensors_80.O_80_Part_Stuck == true && ...
        | Status2c_10 == true]
    Distribution_Counted.PistonStartsMoveBackward -> Distribution_Counted.ArmToMagazine : [Sensors_80.O_80_Pist_Bck == true && ...
        | Status2c_7 == true]
    Distribution_Counted.ArmToDelivery -> Distribution_Counted.ArmCloseDelivery : [Sensors_80.O_80_Arm_Mag == false &&...
        | Status2c_2 == true]
    Distribution_Counted.ArmToMagazine -> Distribution_Counted.ArmCloseDeliver1 : [Sensors_80.O_80_Arm_Del == false &&...
        | Status2c_8 == true]
    Distribution_Counted.ArmCloseDeliver1 -> Distribution_Counted.ArmArrives_PicksPart : [Sensors_80.O_80_Arm_Mag == true && ...
        | Status2c_9 == true]
    Distribution_Counted.PartFed -> Distribution_Counted.PistonStartsMoveBackward : [Status2c_6 == true]
    (default) -> Distribution_Counted.InitialCondition
    Distribution_Counted.ArmToDelivery1 -> Distribution_Counted.ArmCloseDelivery2 : [Sensors_80.O_80_Arm_Mag == false &&...
        | Status2c_11 == true]
    (junction 804) -> Distribution_Counted.ArmArrives_FeedsPart
    (junction 820) -> (junction 804)
    Distribution_Counted.PartDel_CheckLoop -> (junction 821) [order 1] : [LoopDistCont == true]
    Distribution_Counted.PartDel_CheckLoop -> Distribution_Counted.T1 [order 3] : after(4,sec)
    (junction 821) -> (junction 820)
  note: Conveyor
  state SRB Output
    state ArmToMagazine1
      entry:
      Status2c_14 = false;
      during:
      Actuators_80.F_82_Suction_Off;
      Actuators_80.F_82_Arm_2_Mag;
      Actuators_80.F_83_Led_Extra1;
      Control_80.C_85_Part_Del;
      if ~Actuators_80.F_82_Suction_Off && ...
      Actuators_80.F_82_Arm_2_Mag && ...
      Actuators_80.F_83_Led_Extra1 && ...
      Control_80.C_85_Part_Del
      Status2c_14 = true;
      else
      Status2c_14 = false;
      end
    state ArmCloseDeliver3
      entry:
      Status2c_15 = false;
      during:
      Sensors_70.O_70_SStation;
      if Sensors_70.O_70_SStation
      Status2c_15 = true;
      else
      Status2c_15 = false;
      end
    state ArmArrives_Finish
      entry:
      Status2c_16 = false;
      during:
      Actuators_80.F_82_Arm_2_Mag;
      if ~Actuators_80.F_82_Arm_2_Mag;
      Status2c_16 = true;
      else
      Status2c_16 = false;
      end
    state ArmToMagazine
      entry:
      Status2c_8 = false;
      during:
      Actuators_80.F_82_Arm_2_Mag;
      if Actuators_80.F_82_Arm_2_Mag
      Status2c_8 = true;
      else
      Status2c_8 = false;
      end
    state ArmCloseDeliver1
      entry:
      Status2c_9 = false;
      during:
      Sensors_70.O_70_SStation;
      if Sensors_70.O_70_SStation
      Status2c_9 = true;
      else
      Status2c_9 = false;
      end
    state ArmArrives_PicksPart
      entry:
      Status2c_10 = false;
      during:
      Actuators_80.F_82_Suction_On;
      Actuators_80.F_82_Arm_2_Mag;
      if Actuators_80.F_82_Suction_On && ...
      ~Actuators_80.F_82_Arm_2_Mag
      Status2c_10 = true;
      else
      Status2c_10 = false;
      end
    state ArmToDelivery1
      entry:
      Status2c_11 = false;
      during:
      Actuators_80.F_82_Arm_2_Del
      if Actuators_80.F_82_Arm_2_Del
      Status2c_11 = true;
      else
      Status2c_11 = false;
      end
    state ArmCloseDelivery2
      entry:
      Status2c_12 = false;
      during:
      Sensors_70.O_70_SStation;
      if Sensors_70.O_70_SStation
      Status2c_12 = true;
      else
      Status2c_12 = false;
      end
    state ArmArrives_DeliversPart
      entry:
      Status2c_13 = false;
      during:
      Actuators_80.F_82_Suction_On;
      Actuators_80.F_82_Suction_Off;
      Actuators_80.F_82_Arm_2_Del;
      if ~Actuators_80.F_82_Suction_On && ...
      Actuators_80.F_82_Suction_Off && ...
      ~Actuators_80.F_82_Arm_2_Del
      Status2c_13 = true;
      else
      Status2c_13 = false;
      end
    state PartDel_CheckLoop
      entry:
      LoopDistCont = false;
      during:
      Control_80.C_85_Part_Del
      Control_80.C_87_RQ_MParts
      if Control_80.C_85_Part_Del && ...
      Control_80.C_87_RQ_MParts == 0
      LoopDistCont = true;
      else
      LoopDistCont = false;
      end
    state InitialCondition
      entry:
      Status2c_1 = false;
      during:
      Control_80.C_85_Initialization;
      Control_80.C_86_Mag_Parts;
      Control_80.C_82_Profibus;
      Control_80.C_85_Continuous;
      Sensors_80.O_80_Arm_Mag;
      Sensors_80.O_81_Key_Pos;
      if Control_80.C_85_Initialization&& ...
      Control_80.C_86_Mag_Parts ~= 0 && ...
      Control_80.C_82_Profibus && ...
      Control_80.C_85_Continuous && ...
      Sensors_80.O_80_Arm_Mag && ...
      Sensors_80.O_81_Key_Pos
      Status2c_1 = true;
      else
      Status2c_1 = false;
      end
    state ArmToDelivery
      entry:
      Status2c_2 = false;
      during:
      Actuators_80.F_82_Arm_2_Del
      if Actuators_80.F_82_Arm_2_Del
      Status2c_2 = true;
      else
      Status2c_2 = false;
      end
    state ArmCloseDelivery
      entry:
      Status2c_3 = false;
      during:
      Sensors_70.O_70_SStation;
      if Sensors_70.O_70_SStation
      Status2c_3 = true;
      else
      Status2c_3 = false;
      end
    state ArmArrives_FeedsPart
      entry:
      Status2b_4 = false;
      during:
      Actuators_80.F_82_Pist_Adv;
      Actuators_80.F_82_Arm_2_Del;
      if Actuators_80.F_82_Pist_Adv && ...
      ~Actuators_80.F_82_Arm_2_Del
      Status2b_4 = true;
      else
      Status2b_4 = false;
      end
    state PistonStartsMoveForward
      entry:
      Status2c_5 = false;
      during:
      Sensors_80.O_80_Pist_Bck;
      if ~Sensors_80.O_80_Pist_Bck
      Status2c_5 = true;
      else
      Status2c_5 = false;
      end
    state PartFed
      entry:
      Status2c_6 = false;
      during:
      Actuators_80.F_82_Pist_Adv;
      if ~Actuators_80.F_82_Pist_Adv
      Status2c_6 = true;
      else
      Status2c_6 = false;
      end
    state PistonStartsMoveBackward
      entry:
      Status2c_7 = false;
      during:
      Sensors_80.O_80_Pist_Fwd;
      if ~Sensors_80.O_80_Pist_Fwd
      Status2c_7 = true;
      else
      Status2c_7 = false;
      end
    state T1
      during:
      Control_80.C_85_Part_Del
      Actuators_80.F_83_Led_Extra1
    SRB.InitialCondition -> SRB.ArmToDelivery : [Sensors_80.O_81_Start == true | ...
        | Control_80.C_85_Start == true | ...
        | Control_70.C_75_RQ_Wrong == true | ...
        | (AS_i_70.A_74_CRoute_In80 == true && Sensors_80.O_81_Key_Pos == true) ]
    SRB.ArmArrives_FeedsPart -> SRB.PistonStartsMoveForward : [Status2b_4 == true]
    SRB.PartDel_CheckLoop -> SRB.ArmToMagazine1 [order 2] : [LoopDistCont == false]
    SRB.ArmCloseDeliver3 -> SRB.ArmArrives_Finish : [Sensors_80.O_80_Arm_Mag == true && ...
        | Status2c_15 == true]
    SRB.ArmCloseDelivery2 -> SRB.ArmArrives_DeliversPart : [Sensors_80.O_80_Arm_Del == true && ...
        | Status2c_12 == true]
    SRB.ArmCloseDelivery -> SRB.ArmArrives_FeedsPart : [Sensors_80.O_80_Arm_Del == true && ...
        | Status2c_3 == true]
    SRB.PistonStartsMoveForward -> SRB.PartFed : [Sensors_80.O_80_Pist_Fwd == true && ...
        | Status2c_5 == true]
    SRB.ArmArrives_DeliversPart -> SRB.PartDel_CheckLoop : [Sensors_80.O_80_Part_Stuck == false && ...
        | Status2c_13 == true]
    SRB.ArmToMagazine1 -> SRB.ArmCloseDeliver3 : [Sensors_80.O_80_Arm_Del == false &&...
        | Status2c_14 == true]
    SRB.ArmArrives_PicksPart -> SRB.ArmToDelivery1 : [Sensors_80.O_80_Part_Stuck == true && ...
        | Status2c_10 == true]
    SRB.PistonStartsMoveBackward -> SRB.ArmToMagazine : [Sensors_80.O_80_Pist_Bck == true && ...
        | Status2c_7 == true]
    SRB.ArmToDelivery -> SRB.ArmCloseDelivery : [Sensors_80.O_80_Arm_Mag == false &&...
        | Status2c_2 == true]
    SRB.ArmToMagazine -> SRB.ArmCloseDeliver1 : [Sensors_80.O_80_Arm_Del == false &&...
        | Status2c_8 == true]
    SRB.ArmCloseDeliver1 -> SRB.ArmArrives_PicksPart : [Sensors_80.O_80_Arm_Mag == true && ...
        | Status2c_9 == true]
    SRB.PartFed -> SRB.PistonStartsMoveBackward : [Status2c_6 == true]
    (default) -> SRB.InitialCondition
    SRB.ArmToDelivery1 -> SRB.ArmCloseDelivery2 : [Sensors_80.O_80_Arm_Mag == false &&...
        | Status2c_11 == true]
    (junction 2369) -> SRB.ArmArrives_FeedsPart
    (junction 2348) -> (junction 2369)
    SRB.PartDel_CheckLoop -> (junction 2361) [order 1] : [LoopDistCont == true]
    SRB.PartDel_CheckLoop -> SRB.T1 [order 3] : after(4,sec)
    (junction 2361) -> (junction 2348)
  state CartToProcessing4
    state InitialCondition
      entry:
      Status4_1 = false;
      during:
      Actuators_20.F_22_Conveyor;
      AS_i_70.A_74_Cart_Full;
      AS_i_70.A_73_TestCartID;
      AS_i_70.A_74_Pist_Bck;
      AS_i_70.A_74_Release_FB;
      if ~Actuators_20.F_22_Conveyor && ...
      AS_i_70.A_74_Cart_Full && ...
      ~AS_i_70.A_73_TestCartID ~= 0 && ...
      ~AS_i_70.A_74_Pist_Bck && ...
      ~AS_i_70.A_74_Release_FB
      Status4_1 = true;
      else
      Status4_1 = false;
      end
    state StartsProcess
      entry:
      Status4_2 = false;
      during:
      Actuators_20.F_22_Conveyor;
      AS_i_70.A_73_TestCartID;
      AS_i_70.A_74_Pist_Bck;
      AS_i_70.A_74_Release_FB;
      if Actuators_20.F_22_Conveyor && ...
      AS_i_70.A_73_TestCartID == 0 && ...
      AS_i_70.A_74_Pist_Bck && ...
      AS_i_70.A_74_Release_FB
      Status4_2 = true;
      else
      Status4_2 = false;
      end
    state PartLeavesSensor
      entry:
      Status4_3 = false;
      during:
      Actuators_70.F_73_Led_Extra2;
      AS_i_70.A_74_Cart_Full;
      AS_i_70.A_74_Optic;
      if ~Actuators_70.F_73_Led_Extra2 && ...
      ~AS_i_70.A_74_Cart_Full && ...
      ~AS_i_70.A_74_Optic
      Status4_3 = true;
      else
      Status4_3 = false;
      end
    state CartStartsMoving
      entry:
      Status4_4 = false;
      during:
      Actuators_70.F_73_Led_Extra1;
      AS_i_70.A_74_No_Cart;
      AS_i_70.A_74_Cart_Stat;
      if Actuators_70.F_73_Led_Extra1 && ...
      AS_i_70.A_74_No_Cart && ...
      ~AS_i_70.A_74_Cart_Stat
      Status4_4 = true;
      else
      Status4_4 = false;
      end
    state CartGetsNearNextStation
      entry:
      Status4_5 = false;
      during:
      AS_i_70.A_74_Cart_Next;
      AS_i_70.A_74_Pist_Bck;
      AS_i_70.A_74_Release_FB;
      if AS_i_70.A_74_Cart_Next && ...
      ~AS_i_70.A_74_Pist_Bck && ...
      ~AS_i_70.A_74_Release_FB
      Status4_5 = true;
      else
      Status4_5 = false;
      end
    state DetectionofCartNumberinStation
      entry:
      Status4_6 = false;
      during:
      AS_i_90.A_93_ProcCartID
      if ~AS_i_90.A_93_ProcCartID ~=0
      Status4_6 = true;
      else
      Status4_6 = false;
      end
    state CartPassesNextStation
      entry:
      Status4_7 = false;
      during:
      AS_i_70.A_74_Cart_Next
      if ~AS_i_70.A_74_Cart_Next
      Status4_7 = true;
      else
      Status4_7 = false;
      end
    state PartArrivesSensor
      entry:
      Status4_8 = false;
      during:
      AS_i_90.A_94_Optic;
      if AS_i_90.A_94_Optic
      Status4_8 = true;
      else
      Status4_8 = false;
      end
    state CartArrivesinNextStation
      entry:
      Status4_9 = false;
      during:
      Control_20.C_25_CartDel;
      Actuators_90.F_93_Led_Extra1;
      AS_i_90.A_94_Cart_Stat;
      AS_i_90.A_94_No_Cart;
      AS_i_90.A_94_Cart_Full;
      AS_i_90.A_94_CRoute_In;
      if Control_20.C_25_CartDel && ...
      ~Actuators_90.F_93_Led_Extra1 && ...
      AS_i_90.A_94_Cart_Stat && ...
      ~AS_i_90.A_94_No_Cart && ...
      AS_i_90.A_94_Cart_Full && ...
      AS_i_90.A_94_CRoute_In
      Status4_9 = true;
      else
      Status4_9 = false;
      end
    state T1
      during:
      Control_20.C_25_Request
    state T3
      during:
      Control_20.C_25_CartDel
    state T2
      during:
      AS_i_90.A_94_CRoute_In
    (default) -> CartToProcessing4.InitialCondition
    CartToProcessing4.DetectionofCartNumberinStation -> CartToProcessing4.CartPassesNextStation : [Sensors_20.O_24_Cart_Next == false && ...
        | Status4_6 == true]
    CartToProcessing4.InitialCondition -> CartToProcessing4.StartsProcess : [Control_20.C_25_Request == true && ...
        |  Status4_1 == true]
    CartToProcessing4.StartsProcess -> CartToProcessing4.PartLeavesSensor [order 1] : [Sensors_20.O_24_Optic == false && ...
        | Status4_2 == true]
    CartToProcessing4.PartLeavesSensor -> CartToProcessing4.CartStartsMoving : [Sensors_20.O_24_Cart_Stat == false && ...
        | Status4_3 == true]
    CartToProcessing4.CartStartsMoving -> CartToProcessing4.CartGetsNearNextStation : [Sensors_20.O_24_Cart_Next == true && ...
        | Status4_4 == true]
    CartToProcessing4.CartGetsNearNextStation -> CartToProcessing4.DetectionofCartNumberinStation : [Sensors_20.O_24_Count == true && ...
        | Status4_5 == true]
    CartToProcessing4.CartPassesNextStation -> CartToProcessing4.PartArrivesSensor : [Sensors_20.O_25_Optic == true && ...
        | Status4_7 == true]
    CartToProcessing4.PartArrivesSensor -> CartToProcessing4.CartArrivesinNextStation : [Sensors_20.O_25_Cart_Stat == true && ...
        | Status4_8 == true]
    CartToProcessing4.StartsProcess -> CartToProcessing4.T1 [order 2] : [after(2, sec)]
    CartToProcessing4.CartArrivesinNextStation -> (junction 2095)
    (junction 2095) -> CartToProcessing4.T3 [order 2] : [after(3,sec)]
    (junction 2095) -> CartToProcessing4.T2 [order 1] : [after(2,sec)]
  note: Conveyor
  note: Processing [100]
  state CartToProcessing
    state InitialCondition
      entry:
      Status4_1 = false;
      during:
      Actuators_20.F_22_Conveyor;
      AS_i_70.A_74_Cart_Full;
      AS_i_70.A_73_TestCartID;
      AS_i_70.A_74_Pist_Bck;
      AS_i_70.A_74_Release_FB;
      if ~Actuators_20.F_22_Conveyor && ...
      AS_i_70.A_74_Cart_Full && ...
      ~AS_i_70.A_73_TestCartID ~= 0 && ...
      ~AS_i_70.A_74_Pist_Bck && ...
      ~AS_i_70.A_74_Release_FB
      Status4_1 = true;
      else
      Status4_1 = false;
      end
    state StartsProcess
      entry:
      Status4_2 = false;
      during:
      Actuators_20.F_22_Conveyor;
      AS_i_70.A_73_TestCartID;
      AS_i_70.A_74_Pist_Bck;
      AS_i_70.A_74_Release_FB;
      if Actuators_20.F_22_Conveyor && ...
      AS_i_70.A_73_TestCartID == 0 && ...
      AS_i_70.A_74_Pist_Bck && ...
      AS_i_70.A_74_Release_FB
      Status4_2 = true;
      else
      Status4_2 = false;
      end
    state PartLeavesSensor
      entry:
      Status4_3 = false;
      during:
      Actuators_70.F_73_Led_Extra2;
      AS_i_70.A_74_Cart_Full;
      AS_i_70.A_74_Optic;
      if ~Actuators_70.F_73_Led_Extra2 && ...
      ~AS_i_70.A_74_Cart_Full && ...
      ~AS_i_70.A_74_Optic
      Status4_3 = true;
      else
      Status4_3 = false;
      end
    state CartStartsMoving
      entry:
      Status4_4 = false;
      during:
      Actuators_70.F_73_Led_Extra1;
      AS_i_70.A_74_No_Cart;
      AS_i_70.A_74_Cart_Stat;
      if Actuators_70.F_73_Led_Extra1 && ...
      AS_i_70.A_74_No_Cart && ...
      ~AS_i_70.A_74_Cart_Stat
      Status4_4 = true;
      else
      Status4_4 = false;
      end
    state CartGetsNearNextStation
      entry:
      Status4_5 = false;
      during:
      AS_i_70.A_74_Cart_Next;
      AS_i_70.A_74_Pist_Bck;
      AS_i_70.A_74_Release_FB;
      if AS_i_70.A_74_Cart_Next && ...
      ~AS_i_70.A_74_Pist_Bck && ...
      ~AS_i_70.A_74_Release_FB
      Status4_5 = true;
      else
      Status4_5 = false;
      end
    state DetectionofCartNumberinStation
      entry:
      Status4_6 = false;
      during:
      AS_i_90.A_93_ProcCartID
      if ~AS_i_90.A_93_ProcCartID ~=0
      Status4_6 = true;
      else
      Status4_6 = false;
      end
    state CartPassesNextStation
      entry:
      Status4_7 = false;
      during:
      AS_i_70.A_74_Cart_Next
      if ~AS_i_70.A_74_Cart_Next
      Status4_7 = true;
      else
      Status4_7 = false;
      end
    state PartArrivesSensor
      entry:
      Status4_8 = false;
      during:
      AS_i_90.A_94_Optic;
      if AS_i_90.A_94_Optic
      Status4_8 = true;
      else
      Status4_8 = false;
      end
    state CartArrivesinNextStation
      entry:
      Status4_9 = false;
      during:
      Control_20.C_25_CartDel;
      Actuators_90.F_93_Led_Extra1;
      AS_i_90.A_94_Cart_Stat;
      AS_i_90.A_94_No_Cart;
      AS_i_90.A_94_Cart_Full;
      AS_i_90.A_94_CRoute_In;
      if Control_20.C_25_CartDel && ...
      ~Actuators_90.F_93_Led_Extra1 && ...
      AS_i_90.A_94_Cart_Stat && ...
      ~AS_i_90.A_94_No_Cart && ...
      AS_i_90.A_94_Cart_Full && ...
      AS_i_90.A_94_CRoute_In
      Status4_9 = true;
      else
      Status4_9 = false;
      end
    state T1
      during:
      Control_20.C_25_Request
    state T3
      during:
      Control_20.C_25_CartDel
    state T2
      during:
      AS_i_90.A_94_CRoute_In
    (default) -> CartToProcessing.InitialCondition
    CartToProcessing.DetectionofCartNumberinStation -> CartToProcessing.CartPassesNextStation : [Sensors_20.O_24_Cart_Next == false && ...
        | Status4_6 == true]
    CartToProcessing.InitialCondition -> CartToProcessing.StartsProcess : [Control_20.C_25_Request == true && ...
        |  Status4_1 == true]
    CartToProcessing.StartsProcess -> CartToProcessing.PartLeavesSensor [order 1] : [Sensors_20.O_24_Optic == false && ...
        | Status4_2 == true]
    CartToProcessing.PartLeavesSensor -> CartToProcessing.CartStartsMoving : [Sensors_20.O_24_Cart_Stat == false && ...
        | Status4_3 == true]
    CartToProcessing.CartStartsMoving -> CartToProcessing.CartGetsNearNextStation : [Sensors_20.O_24_Cart_Next == true && ...
        | Status4_4 == true]
    CartToProcessing.CartGetsNearNextStation -> CartToProcessing.DetectionofCartNumberinStation : [Sensors_20.O_24_Count == true && ...
        | Status4_5 == true]
    CartToProcessing.CartPassesNextStation -> CartToProcessing.PartArrivesSensor : [Sensors_20.O_25_Optic == true && ...
        | Status4_7 == true]
    CartToProcessing.PartArrivesSensor -> CartToProcessing.CartArrivesinNextStation : [Sensors_20.O_25_Cart_Stat == true && ...
        | Status4_8 == true]
    CartToProcessing.StartsProcess -> CartToProcessing.T1 [order 2] : [after(2, sec)]
    CartToProcessing.CartArrivesinNextStation -> (junction 1033)
    (junction 1033) -> CartToProcessing.T3 [order 2] : [after(3,sec)]
    (junction 1033) -> CartToProcessing.T2 [order 1] : [after(2,sec)]
  state Distribution_Single1
    state PistonStartsMoveBackward
      entry:
      Status2a_7 = false;
      during:
      Sensors_80.O_80_Pist_Fwd;
      if ~Sensors_80.O_80_Pist_Fwd
      Status2a_7 = true;
      else
      Status2a_7 = false;
      end
    state PartFed
      entry:
      Status2a_6 = false;
      during:
      Actuators_80.F_82_Pist_Adv;
      if ~Actuators_80.F_82_Pist_Adv
      Status2a_6 = true;
      else
      Status2a_6 = false;
      end
    state ArmToMagazine
      entry:
      Status2a_8 = false;
      during:
      Actuators_80.F_82_Arm_2_Mag;
      if Actuators_80.F_82_Arm_2_Mag
      Status2a_8 = true;
      else
      Status2a_8 = false;
      end
    state ArmCloseDeliver1
      entry:
      Status2a_9 = false;
      during:
      Sensors_70.O_70_SStation;
      if Sensors_70.O_70_SStation
      Status2a_9 = true;
      else
      Status2a_9 = false;
      end
    state ArmArrives_PicksPart
      entry:
      Status2a_10 = false;
      during:
      Actuators_80.F_82_Suction_On;
      Actuators_80.F_82_Arm_2_Mag;
      if Actuators_80.F_82_Suction_On && ...
      ~Actuators_80.F_82_Arm_2_Mag
      Status2a_10 = true;
      else
      Status2a_10 = false;
      end
    state ArmToDelivery1
      entry:
      Status2a_11 = false;
      during:
      Actuators_80.F_82_Arm_2_Del
      if Actuators_80.F_82_Arm_2_Del
      Status2a_11 = true;
      else
      Status2a_11 = false;
      end
    state ArmCloseDelivery2
      entry:
      Status2a_12 = false;
      during:
      Sensors_70.O_70_SStation;
      if Sensors_70.O_70_SStation
      Status2a_12 = true;
      else
      Status2a_12 = false;
      end
    state ArmArrives_DeliversPart
      entry:
      Status2a_13 = false;
      during:
      Actuators_80.F_82_Suction_On;
      Actuators_80.F_82_Suction_Off;
      Actuators_80.F_82_Arm_2_Del;
      if ~Actuators_80.F_82_Suction_On && ...
      Actuators_80.F_82_Suction_Off && ...
      ~Actuators_80.F_82_Arm_2_Del
      Status2a_13 = true;
      else
      Status2a_13 = false;
      end
    state ArmToMagazine1
      entry:
      Status2a_14 = false;
      during:
      Actuators_80.F_82_Suction_Off;
      Actuators_80.F_82_Arm_2_Mag;
      Actuators_80.F_83_Led_Extra1;
      Control_80.C_85_Part_Del;
      if ~Actuators_80.F_82_Suction_Off && ...
      Actuators_80.F_82_Arm_2_Mag && ...
      Actuators_80.F_83_Led_Extra1 && ...
      Control_80.C_85_Part_Del
      Status2a_14 = true;
      else
      Status2a_14 = false;
      end
    state ArmCloseDeliver3
      entry:
      Status2a_15 = false;
      during:
      Sensors_70.O_70_SStation;
      if Sensors_70.O_70_SStation
      Status2a_15 = true;
      else
      Status2a_15 = false;
      end
    state ArmArrives_Finish
      entry:
      Status2a_16 = false;
      during:
      Actuators_80.F_82_Arm_2_Mag;
      if ~Actuators_80.F_82_Arm_2_Mag;
      Status2a_16 = true;
      else
      Status2a_16 = false;
      end
    state InitialCondition
      entry:
      Status2a_1 = false;
      during:
      Control_80.C_85_Initialization;
      Control_80.C_86_Mag_Parts;
      Control_80.C_82_Profibus;
      Control_80.C_85_Single;
      Sensors_80.O_80_Arm_Mag;
      Sensors_80.O_81_Key_Pos;
      if Control_80.C_85_Initialization&& ...
      Control_80.C_86_Mag_Parts ~= 0 && ...
      Control_80.C_82_Profibus && ...
      Control_80.C_85_Single && ...
      Sensors_80.O_80_Arm_Mag && ...
      Sensors_80.O_81_Key_Pos
      Status2a_1 = true;
      else
      Status2a_1 = false;
      end
    state ArmToDelivery
      entry:
      Status2a_2 = false;
      during:
      Actuators_80.F_82_Arm_2_Del;
      if Actuators_80.F_82_Arm_2_Del
      Status2a_2 = true;
      else
      Status2a_2 = false;
      end
    state ArmCloseDelivery
      entry:
      Status2a_3 = false;
      during:
      Sensors_70.O_70_SStation;
      if Sensors_70.O_70_SStation
      Status2a_3 = true;
      else
      Status2a_3 = false;
      end
    state ArmArrives_FeedsPart
      entry:
      Status2a_4 = false;
      during:
      Actuators_80.F_82_Pist_Adv;
      Actuators_80.F_82_Arm_2_Del;
      if Actuators_80.F_82_Pist_Adv && ...
      ~Actuators_80.F_82_Arm_2_Del
      Status2a_4 = true;
      else
      Status2a_4 = false;
      end
    state PistonStartsMoveForward
      entry:
      Status2a_5 = false;
      during:
      Sensors_80.O_80_Pist_Bck;
      if ~Sensors_80.O_80_Pist_Bck
      Status2a_5 = true;
      else
      Status2a_5 = false;
      end
    state T1
      during:
      Control_80.C_85_Part_Del
      Actuators_80.F_83_Led_Extra1
    (default) -> Distribution_Single1.InitialCondition
    Distribution_Single1.ArmToMagazine1 -> (junction 1690)
    (junction 1690) -> Distribution_Single1.ArmCloseDeliver3 [order 1] : [Sensors_80.O_80_Arm_Del == false &&...
        |  Status2a_14 == true]
    Distribution_Single1.ArmToDelivery -> Distribution_Single1.ArmCloseDelivery : [Sensors_80.O_80_Arm_Mag == false &&...
        |  Status2a_2 == true]
    Distribution_Single1.ArmCloseDelivery -> Distribution_Single1.ArmArrives_FeedsPart : [Sensors_80.O_80_Arm_Del == true && ...
        | Status2a_3 == true]
    Distribution_Single1.ArmArrives_DeliversPart -> Distribution_Single1.ArmToMagazine1 : [Sensors_80.O_80_Part_Stuck == false && ...
        | Status2a_13 == true]
    Distribution_Single1.ArmCloseDelivery2 -> Distribution_Single1.ArmArrives_DeliversPart : [Sensors_80.O_80_Arm_Del == true && ...
        | Status2a_12 == true]
    Distribution_Single1.ArmArrives_FeedsPart -> Distribution_Single1.PistonStartsMoveForward : [Status2a_4 == true]
    Distribution_Single1.PistonStartsMoveBackward -> Distribution_Single1.ArmToMagazine : [Sensors_80.O_80_Pist_Bck == true && ...
        | Status2a_7 == true]
    Distribution_Single1.ArmCloseDeliver1 -> Distribution_Single1.ArmArrives_PicksPart : [Sensors_80.O_80_Arm_Mag == true && ...
        | Status2a_9 == true]
    Distribution_Single1.PartFed -> Distribution_Single1.PistonStartsMoveBackward : [Status2a_6 == true]
    Distribution_Single1.ArmToMagazine -> Distribution_Single1.ArmCloseDeliver1 : [Sensors_80.O_80_Arm_Del == false &&...
        | Status2a_8 == true]
    Distribution_Single1.InitialCondition -> Distribution_Single1.ArmToDelivery : [Sensors_80.O_81_Start == true | ...
        | Control_80.C_85_Start == true | ...
        | Control_70.C_75_RQ_Wrong == true | ...
        | (AS_i_70.A_74_CRoute_In80 == true && Sensors_80.O_81_Key_Pos == true) ]
    Distribution_Single1.ArmCloseDeliver3 -> Distribution_Single1.ArmArrives_Finish : [Sensors_80.O_80_Arm_Mag == true && ...
        | Status2a_15 == true]
    Distribution_Single1.ArmToDelivery1 -> Distribution_Single1.ArmCloseDelivery2 : [Sensors_80.O_80_Arm_Mag == false &&...
        | Status2a_11 == true]
    Distribution_Single1.PistonStartsMoveForward -> Distribution_Single1.PartFed : [Sensors_80.O_80_Pist_Fwd == true && ...
        | Status2a_5 == true]
    Distribution_Single1.ArmArrives_PicksPart -> Distribution_Single1.ArmToDelivery1 : [Sensors_80.O_80_Part_Stuck == true && ...
        | Status2a_10 == true]
    (junction 1690) -> (junction 1704) [order 2] : after(4,sec)
    (junction 1704) -> Distribution_Single1.T1
  state SRB1 Output
    state ArmToMagazine1
      entry:
      Status2c_14 = false;
      during:
      Actuators_80.F_82_Suction_Off;
      Actuators_80.F_82_Arm_2_Mag;
      Actuators_80.F_83_Led_Extra1;
      Control_80.C_85_Part_Del;
      if ~Actuators_80.F_82_Suction_Off && ...
      Actuators_80.F_82_Arm_2_Mag && ...
      Actuators_80.F_83_Led_Extra1 && ...
      Control_80.C_85_Part_Del
      Status2c_14 = true;
      else
      Status2c_14 = false;
      end
    state ArmCloseDeliver3
      entry:
      Status2c_15 = false;
      during:
      Sensors_70.O_70_SStation;
      if Sensors_70.O_70_SStation
      Status2c_15 = true;
      else
      Status2c_15 = false;
      end
    state ArmArrives_Finish
      entry:
      Status2c_16 = false;
      during:
      Actuators_80.F_82_Arm_2_Mag;
      if ~Actuators_80.F_82_Arm_2_Mag;
      Status2c_16 = true;
      else
      Status2c_16 = false;
      end
    state ArmToMagazine
      entry:
      Status2c_8 = false;
      during:
      Actuators_80.F_82_Arm_2_Mag;
      if Actuators_80.F_82_Arm_2_Mag
      Status2c_8 = true;
      else
      Status2c_8 = false;
      end
    state ArmCloseDeliver1
      entry:
      Status2c_9 = false;
      during:
      Sensors_70.O_70_SStation;
      if Sensors_70.O_70_SStation
      Status2c_9 = true;
      else
      Status2c_9 = false;
      end
    state ArmArrives_PicksPart
      entry:
      Status2c_10 = false;
      during:
      Actuators_80.F_82_Suction_On;
      Actuators_80.F_82_Arm_2_Mag;
      if Actuators_80.F_82_Suction_On && ...
      ~Actuators_80.F_82_Arm_2_Mag
      Status2c_10 = true;
      else
      Status2c_10 = false;
      end
    state ArmToDelivery1
      entry:
      Status2c_11 = false;
      during:
      Actuators_80.F_82_Arm_2_Del
      if Actuators_80.F_82_Arm_2_Del
      Status2c_11 = true;
      else
      Status2c_11 = false;
      end
    state ArmCloseDelivery2
      entry:
      Status2c_12 = false;
      during:
      Sensors_70.O_70_SStation;
      if Sensors_70.O_70_SStation
      Status2c_12 = true;
      else
      Status2c_12 = false;
      end
    state ArmArrives_DeliversPart
      entry:
      Status2c_13 = false;
      during:
      Actuators_80.F_82_Suction_On;
      Actuators_80.F_82_Suction_Off;
      Actuators_80.F_82_Arm_2_Del;
      if ~Actuators_80.F_82_Suction_On && ...
      Actuators_80.F_82_Suction_Off && ...
      ~Actuators_80.F_82_Arm_2_Del
      Status2c_13 = true;
      else
      Status2c_13 = false;
      end
    state PartDel_CheckLoop
      entry:
      LoopDistCont = false;
      during:
      Control_80.C_85_Part_Del
      Control_80.C_87_RQ_MParts
      if Control_80.C_85_Part_Del && ...
      Control_80.C_87_RQ_MParts == 0
      LoopDistCont = true;
      else
      LoopDistCont = false;
      end
    state InitialCondition
      entry:
      Status2c_1 = false;
      during:
      Control_80.C_85_Initialization;
      Control_80.C_86_Mag_Parts;
      Control_80.C_82_Profibus;
      Control_80.C_85_Continuous;
      Sensors_80.O_80_Arm_Mag;
      Sensors_80.O_81_Key_Pos;
      if Control_80.C_85_Initialization&& ...
      Control_80.C_86_Mag_Parts ~= 0 && ...
      Control_80.C_82_Profibus && ...
      Control_80.C_85_Continuous && ...
      Sensors_80.O_80_Arm_Mag && ...
      Sensors_80.O_81_Key_Pos
      Status2c_1 = true;
      else
      Status2c_1 = false;
      end
    state ArmToDelivery
      entry:
      Status2c_2 = false;
      during:
      Actuators_80.F_82_Arm_2_Del
      if Actuators_80.F_82_Arm_2_Del
      Status2c_2 = true;
      else
      Status2c_2 = false;
      end
    state ArmCloseDelivery
      entry:
      Status2c_3 = false;
      during:
      Sensors_70.O_70_SStation;
      if Sensors_70.O_70_SStation
      Status2c_3 = true;
      else
      Status2c_3 = false;
      end
    state ArmArrives_FeedsPart
      entry:
      Status2b_4 = false;
      during:
      Actuators_80.F_82_Pist_Adv;
      Actuators_80.F_82_Arm_2_Del;
      if Actuators_80.F_82_Pist_Adv && ...
      ~Actuators_80.F_82_Arm_2_Del
      Status2b_4 = true;
      else
      Status2b_4 = false;
      end
    state PistonStartsMoveForward
      entry:
      Status2c_5 = false;
      during:
      Sensors_80.O_80_Pist_Bck;
      if ~Sensors_80.O_80_Pist_Bck
      Status2c_5 = true;
      else
      Status2c_5 = false;
      end
    state PartFed
      entry:
      Status2c_6 = false;
      during:
      Actuators_80.F_82_Pist_Adv;
      if ~Actuators_80.F_82_Pist_Adv
      Status2c_6 = true;
      else
      Status2c_6 = false;
      end
    state PistonStartsMoveBackward
      entry:
      Status2c_7 = false;
      during:
      Sensors_80.O_80_Pist_Fwd;
      if ~Sensors_80.O_80_Pist_Fwd
      Status2c_7 = true;
      else
      Status2c_7 = false;
      end
    state T1
      during:
      Control_80.C_85_Part_Del
      Actuators_80.F_83_Led_Extra1
    SRB1.InitialCondition -> SRB1.ArmToDelivery : [Sensors_80.O_81_Start == true | ...
        | Control_80.C_85_Start == true | ...
        | Control_70.C_75_RQ_Wrong == true | ...
        | (AS_i_70.A_74_CRoute_In80 == true && Sensors_80.O_81_Key_Pos == true) ]
    SRB1.ArmArrives_FeedsPart -> SRB1.PistonStartsMoveForward : [Status2b_4 == true]
    SRB1.PartDel_CheckLoop -> SRB1.ArmToMagazine1 [order 2] : [LoopDistCont == false]
    SRB1.ArmCloseDeliver3 -> SRB1.ArmArrives_Finish : [Sensors_80.O_80_Arm_Mag == true && ...
        | Status2c_15 == true]
    SRB1.ArmCloseDelivery2 -> SRB1.ArmArrives_DeliversPart : [Sensors_80.O_80_Arm_Del == true && ...
        | Status2c_12 == true]
    SRB1.ArmCloseDelivery -> SRB1.ArmArrives_FeedsPart : [Sensors_80.O_80_Arm_Del == true && ...
        | Status2c_3 == true]
    SRB1.PistonStartsMoveForward -> SRB1.PartFed : [Sensors_80.O_80_Pist_Fwd == true && ...
        | Status2c_5 == true]
    SRB1.ArmArrives_DeliversPart -> SRB1.PartDel_CheckLoop : [Sensors_80.O_80_Part_Stuck == false && ...
        | Status2c_13 == true]
    SRB1.ArmToMagazine1 -> SRB1.ArmCloseDeliver3 : [Sensors_80.O_80_Arm_Del == false &&...
        | Status2c_14 == true]
    SRB1.ArmArrives_PicksPart -> SRB1.ArmToDelivery1 : [Sensors_80.O_80_Part_Stuck == true && ...
        | Status2c_10 == true]
    SRB1.PistonStartsMoveBackward -> SRB1.ArmToMagazine : [Sensors_80.O_80_Pist_Bck == true && ...
        | Status2c_7 == true]
    SRB1.ArmToDelivery -> SRB1.ArmCloseDelivery : [Sensors_80.O_80_Arm_Mag == false &&...
        | Status2c_2 == true]
    SRB1.ArmToMagazine -> SRB1.ArmCloseDeliver1 : [Sensors_80.O_80_Arm_Del == false &&...
        | Status2c_8 == true]
    SRB1.ArmCloseDeliver1 -> SRB1.ArmArrives_PicksPart : [Sensors_80.O_80_Arm_Mag == true && ...
        | Status2c_9 == true]
    SRB1.PartFed -> SRB1.PistonStartsMoveBackward : [Status2c_6 == true]
    (default) -> SRB1.InitialCondition
    SRB1.ArmToDelivery1 -> SRB1.ArmCloseDelivery2 : [Sensors_80.O_80_Arm_Mag == false &&...
        | Status2c_11 == true]
    (junction 2413) -> SRB1.ArmArrives_FeedsPart
    (junction 2392) -> (junction 2413)
    SRB1.PartDel_CheckLoop -> (junction 2405) [order 1] : [LoopDistCont == true]
    SRB1.PartDel_CheckLoop -> SRB1.T1 [order 3] : after(4,sec)
    (junction 2405) -> (junction 2392)
  note: Handling 2 [90]
  note: Storage [40]
  state Store Par
    state InitialCondition
      entry:
      Status5_1 = false;
      during:
      AS_i_90.A_94_Cart_Full;
      Control_90.C_95_Initialization;
      Control_90.C_95_Cart2Del;
      Control_90.C_92_Profibus;
      Sensors_90.O_91_Key_Pos;
      if AS_i_90.A_94_Cart_Full && ...
      Control_90.C_95_Initialization && ...
      Control_90.C_95_Cart2Del && ...
      Control_90.C_92_Profibus && ...
      Sensors_90.O_91_Key_Pos
      Status5_1 = true;
      else
      Status5_1 = false;
      end
    state FinishesProcess
      entry:
      Status5_13 = false;
      during:
      Control_90.C_95_PD_Proc;
      if Control_90.C_95_PD_Proc
      Status5_13 = true;
      else
      Status5_13 = false;
      end
    (default) -> Store.InitialCondition
    Store.InitialCondition -> ? : [AS_i_90.A_94_CRoute_In == true && ...
        |  Status5_1 == true]
  state PartToProcessing
    state FinishesProcess
      entry:
      Status5_13 = false;
      during:
      Control_90.C_95_PD_Proc;
      if Control_90.C_95_PD_Proc
      Status5_13 = true;
      else
      Status5_13 = false;
      end
    state ClawBeginsAscend
      entry:
      Status5_12 = false;
      during:
      Sensors_90.O_90_Part_in_Claw;
      if ~Sensors_90.O_90_Part_in_Claw
      Status5_12 = true;
      else
      Status5_12 = false;
      end
    state DeliversPart
      entry:
      Status5_11 = false;
      during:
      Actuators_90.F_92_Claw_Down;
      Actuators_90.F_92_Close_Claw;
      if ~Actuators_90.F_92_Claw_Down && ...
      ~Actuators_90.F_92_Close_Claw
      Status5_11 = true;
      else
      Status5_11 = false;
      end
    state ClawDescent
      entry:
      Status5_10 = false;
      during:
      Sensors_90.O_90_Claw_Low;
      Sensors_90.O_90_Claw_High;
      if Sensors_90.O_90_Claw_Low && ...
      ~Sensors_90.O_90_Claw_High
      Status5_10 = true;
      else
      Status5_10 = false;
      end
    state ArmArrives
      entry:
      Status5_9 = false;
      during:
      Actuators_90.F_92_Claw_2_Del;
      Actuators_90.F_92_Claw_Down;
      if ~Actuators_90.F_92_Claw_2_Del && ...
      Actuators_90.F_92_Claw_Down
      Status5_9 = true;
      else
      Status5_9 = false;
      end
    state ArmPassesStorage
      entry:
      Status5_8 = false;
      during:
      Sensors_90.O_90_Claw_Reserve
      if ~Sensors_90.O_90_Claw_Reserve
      Status5_8 = true;
      else
      Status5_8 = false;
      end
    state ArmStartsMovement
      entry:
      Status5_7 = false;
      during:
      Sensors_90.O_90_Claw_Reserve
      if Sensors_90.O_90_Claw_Reserve
      Status5_7 = true;
      else
      Status5_7 = false;
      end
    state ClawFinishesAscend
      entry:
      Status5_6 = false;
      during:
      Actuators_90.F_92_Claw_2_Del;
      if Actuators_90.F_92_Claw_2_Del
      Status5_6 = true;
      else
      Status5_6 = false;
      end
    state PartLeavesCart
      entry:
      Status5_5 = false;
      during:
      AS_i_90.A_94_Cart_Full;
      if ~AS_i_90.A_94_Cart_Full
      Status5_5 = true;
      else
      Status5_5 = false;
      end
    state PartPickup_BeginsAscend
      entry:
      Status5_4 = false;
      during:
      Actuators_90.F_92_Claw_Down;
      Sensors_90.O_90_Claw_Low;
      if ~Actuators_90.F_92_Claw_Down && ...
      ~Sensors_90.O_90_Claw_Low
      Status5_4 = true;
      else
      Status5_4 = false;
      end
    state ClawFinishesDescent
      entry:
      Status5_3 = false;
      during:
      Actuators_90.F_92_Close_Claw;
      if Actuators_90.F_92_Close_Claw
      Status5_3 = true;
      else
      Status5_3 = false;
      end
    state ClawBeginsDescent
      entry:
      Status5_2 = false;
      during:
      Actuators_90.F_92_Claw_Down;
      Control_90.C_95_PD_Proc;
      Control_90.C_95_PD_Cart;
      Sensors_90.O_90_Claw_High;
      if Actuators_90.F_92_Claw_Down && ...
      ~Control_90.C_95_PD_Proc && ...
      ~Control_90.C_95_PD_Cart && ...
      ~Sensors_90.O_90_Claw_High
      Status5_2 = true;
      else
      Status5_2 = false;
      end
    state InitialCondition
      entry:
      Status5_1 = false;
      during:
      AS_i_90.A_94_Cart_Full;
      Control_90.C_95_Initialization;
      Control_90.C_95_Cart2Del;
      Control_90.C_92_Profibus;
      Sensors_90.O_91_Key_Pos;
      if AS_i_90.A_94_Cart_Full && ...
      Control_90.C_95_Initialization && ...
      Control_90.C_95_Cart2Del && ...
      Control_90.C_92_Profibus && ...
      Sensors_90.O_91_Key_Pos
      Status5_1 = true;
      else
      Status5_1 = false;
      end
    (default) -> PartToProcessing.InitialCondition
    PartToProcessing.ArmStartsMovement -> PartToProcessing.ArmPassesStorage : [Sensors_90.O_90_Claw_Reserve == false && ...
        | Status5_7 == true]
    PartToProcessing.ClawBeginsAscend -> PartToProcessing.FinishesProcess : [Sensors_90.O_90_Claw_High == true && ...
        | Status5_12 == true]
    PartToProcessing.DeliversPart -> PartToProcessing.ClawBeginsAscend : [Sensors_90.O_90_Claw_Low && ...
        | Status5_11 == true]
    PartToProcessing.ArmArrives -> PartToProcessing.ClawDescent : [Sensors_90.O_90_Claw_High == false && ...
        | Status5_9 == true]
    PartToProcessing.ClawFinishesAscend -> PartToProcessing.ArmStartsMovement : [Sensors_90.O_90_Claw_Cart == false && ...
        | Status5_6 == true]
    PartToProcessing.ClawFinishesDescent -> PartToProcessing.PartPickup_BeginsAscend : [Sensors_90.O_90_Part_in_Claw == true && ...
        | Status5_3 == true]
    PartToProcessing.PartLeavesCart -> PartToProcessing.ClawFinishesAscend : [Sensors_90.O_90_Claw_High == true && ...
        | Status5_5 == true]
    PartToProcessing.PartPickup_BeginsAscend -> PartToProcessing.PartLeavesCart : [AS_i_90.A_94_Optic == false && ...
        | Status5_4 == true]
    PartToProcessing.ClawDescent -> PartToProcessing.DeliversPart : [Sensors_100.O_100_PInit_Pos == true && ...
        | Status5_10 == true]
    PartToProcessing.ClawBeginsDescent -> PartToProcessing.ClawFinishesDescent : [Sensors_90.O_90_Claw_Low == true && ...
        | Status5_2 == true]
    PartToProcessing.InitialCondition -> PartToProcessing.ClawBeginsDescent : [AS_i_90.A_94_CRoute_In == true && ...
        |  Status5_1 == true]
    PartToProcessing.ArmPassesStorage -> PartToProcessing.ArmArrives : [Sensors_90.O_90_Claw_Del == true && ...
        | Status5_8 == true]
  state Distribution_Continuous1
    state InitialCondition
      entry:
      Status2b_1 = false;
      during:
      Control_80.C_85_Initialization;
      Control_80.C_86_Mag_Parts;
      Control_80.C_82_Profibus;
      Control_80.C_85_Continuous;
      Sensors_80.O_80_Arm_Mag;
      Sensors_80.O_81_Key_Pos;
      if Control_80.C_85_Initialization&& ...
      Control_80.C_86_Mag_Parts ~= 0 && ...
      Control_80.C_82_Profibus && ...
      Control_80.C_85_Continuous && ...
      Sensors_80.O_80_Arm_Mag && ...
      Sensors_80.O_81_Key_Pos
      Status2a_1 = true;
      else
      Status2b_1 = false;
      end
    state ArmToDelivery
      entry:
      Status2b_2 = false;
      during:
      Actuators_80.F_82_Arm_2_Del
      if Actuators_80.F_82_Arm_2_Del
      Status2b_2 = true;
      else
      Status2b_2 = false;
      end
    state ArmCloseDelivery
      entry:
      Status2b_3 = false;
      during:
      Sensors_70.O_70_SStation;
      if Sensors_70.O_70_SStation
      Status2b_3 = true;
      else
      Status2b_3 = false;
      end
    state ArmArrives_FeedsPart
      entry:
      Status2b_4 = false;
      during:
      Actuators_80.F_82_Pist_Adv;
      Actuators_80.F_82_Arm_2_Del;
      if Actuators_80.F_82_Pist_Adv && ...
      ~Actuators_80.F_82_Arm_2_Del
      Status2b_4 = true;
      else
      Status2b_4 = false;
      end
    state PistonStartsMoveForward
      entry:
      Status2b_5 = false;
      during:
      Sensors_80.O_80_Pist_Bck;
      if ~Sensors_80.O_80_Pist_Bck
      Status2b_5 = true;
      else
      Status2b_5 = false;
      end
    state PartFed
      entry:
      Status2b_6 = false;
      during:
      Actuators_80.F_82_Pist_Adv;
      if ~Actuators_80.F_82_Pist_Adv
      Status2b_6 = true;
      else
      Status2b_6 = false;
      end
    state PistonStartsMoveBackward
      entry:
      Status2b_7 = false;
      during:
      Sensors_80.O_80_Pist_Fwd;
      if ~Sensors_80.O_80_Pist_Fwd
      Status2b_7 = true;
      else
      Status2b_7 = false;
      end
    state ArmToMagazine
      entry:
      Status2b_8 = false;
      during:
      Actuators_80.F_82_Arm_2_Mag;
      if Actuators_80.F_82_Arm_2_Mag
      Status2b_8 = true;
      else
      Status2b_8 = false;
      end
    state ArmCloseDeliver1
      entry:
      Status2b_9 = false;
      during:
      Sensors_70.O_70_SStation;
      if Sensors_70.O_70_SStation
      Status2b_9 = true;
      else
      Status2b_9 = false;
      end
    state ArmArrives_PicksPart
      entry:
      Status2b_10 = false;
      during:
      Actuators_80.F_82_Suction_On;
      Actuators_80.F_82_Arm_2_Mag;
      if Actuators_80.F_82_Suction_On && ...
      ~Actuators_80.F_82_Arm_2_Mag
      Status2b_10 = true;
      else
      Status2b_10 = false;
      end
    state ArmToDelivery1
      entry:
      Status2b_11 = false;
      during:
      Actuators_80.F_82_Arm_2_Del
      if Actuators_80.F_82_Arm_2_Del
      Status2b_11 = true;
      else
      Status2b_11 = false;
      end
    state ArmCloseDelivery2
      entry:
      Status2b_12 = false;
      during:
      Sensors_70.O_70_SStation;
      if Sensors_70.O_70_SStation
      Status2b_12 = true;
      else
      Status2b_12 = false;
      end
    state ArmArrives_DeliversPart
      entry:
      Status2b_13 = false;
      during:
      Actuators_80.F_82_Suction_On;
      Actuators_80.F_82_Suction_Off;
      Actuators_80.F_82_Arm_2_Del;
      if ~Actuators_80.F_82_Suction_On && ...
      Actuators_80.F_82_Suction_Off && ...
      ~Actuators_80.F_82_Arm_2_Del
      Status2b_13 = true;
      else
      Status2b_13 = false;
      end
    state PartDel_CheckLoop
      entry:
      LoopDistCont = false;
      during:
      Control_80.C_85_Part_Del
      Control_80.C_86_Mag_Parts
      if Control_80.C_85_Part_Del && ...
      Control_80.C_86_Mag_Parts ~= 0
      LoopDistCont = true;
      else
      LoopDistCont = false;
      end
    state ArmToMagazine1
      entry:
      Status2b_14 = false;
      during:
      Actuators_80.F_82_Suction_Off;
      Actuators_80.F_82_Arm_2_Mag;
      Actuators_80.F_83_Led_Extra1;
      Control_80.C_85_Part_Del;
      if ~Actuators_80.F_82_Suction_Off && ...
      Actuators_80.F_82_Arm_2_Mag && ...
      Actuators_80.F_83_Led_Extra1 && ...
      Control_80.C_85_Part_Del
      Status2b_14 = true;
      else
      Status2b_14 = false;
      end
    state ArmCloseDeliver3
      entry:
      Status2b_15 = false;
      during:
      Sensors_70.O_70_SStation;
      if Sensors_70.O_70_SStation
      Status2b_15 = true;
      else
      Status2b_15 = false;
      end
    state ArmArrives_Finish
      entry:
      Status2b_16 = false;
      during:
      Actuators_80.F_82_Arm_2_Mag;
      if ~Actuators_80.F_82_Arm_2_Mag;
      Status2b_16 = true;
      else
      Status2b_16 = false;
      end
    state T1
      during:
      Control_80.C_85_Part_Del
      Actuators_80.F_83_Led_Extra1
    Distribution_Continuous1.ArmArrives_PicksPart -> Distribution_Continuous1.ArmToDelivery1 : [Sensors_80.O_80_Part_Stuck == true && ...
        | Status2b_10 == true]
    Distribution_Continuous1.ArmArrives_DeliversPart -> Distribution_Continuous1.PartDel_CheckLoop : [Sensors_80.O_80_Part_Stuck == false && ...
        | Status2b_13 == true]
    Distribution_Continuous1.ArmCloseDelivery -> Distribution_Continuous1.ArmArrives_FeedsPart : [Sensors_80.O_80_Arm_Del == true && ...
        | Status2b_3 == true]
    Distribution_Continuous1.ArmArrives_FeedsPart -> Distribution_Continuous1.PistonStartsMoveForward : [Status2b_4 == true]
    (default) -> Distribution_Continuous1.InitialCondition
    Distribution_Continuous1.PartFed -> Distribution_Continuous1.PistonStartsMoveBackward : [Status2b_6 == true]
    Distribution_Continuous1.PistonStartsMoveForward -> Distribution_Continuous1.PartFed : [Sensors_80.O_80_Pist_Fwd == true && ...
        | Status2b_5 == true]
    Distribution_Continuous1.ArmToDelivery -> Distribution_Continuous1.ArmCloseDelivery : [Sensors_80.O_80_Arm_Mag == false &&...
        | Status2a_2 == true]
    Distribution_Continuous1.PistonStartsMoveBackward -> Distribution_Continuous1.ArmToMagazine : [Sensors_80.O_80_Pist_Bck == true && ...
        | Status2b_7 == true]
    Distribution_Continuous1.ArmCloseDelivery2 -> Distribution_Continuous1.ArmArrives_DeliversPart : [Sensors_80.O_80_Arm_Del == true && ...
        | Status2b_12 == true]
    Distribution_Continuous1.ArmToMagazine -> Distribution_Continuous1.ArmCloseDeliver1 : [Sensors_80.O_80_Arm_Del == false &&...
        |  Status2b_8 == true]
    Distribution_Continuous1.ArmCloseDeliver1 -> Distribution_Continuous1.ArmArrives_PicksPart : [Sensors_80.O_80_Arm_Mag == true && ...
        | Status2b_9 == true]
    Distribution_Continuous1.ArmToDelivery1 -> Distribution_Continuous1.ArmCloseDelivery2 : [Sensors_80.O_80_Arm_Mag == false &&...
        |  Status2b_11 == true]
    Distribution_Continuous1.InitialCondition -> Distribution_Continuous1.ArmToDelivery : [Sensors_80.O_81_Start == true | ...
        | Control_80.C_85_Start == true | ...
        | Control_70.C_75_RQ_Wrong == true | ...
        | (AS_i_70.A_74_CRoute_In80 == true && Sensors_80.O_81_Key_Pos == true) ]
    Distribution_Continuous1.ArmToMagazine1 -> Distribution_Continuous1.ArmCloseDeliver3 : [Sensors_80.O_80_Arm_Del == false &&...
        | Status2b_14 == true]
    Distribution_Continuous1.ArmCloseDeliver3 -> Distribution_Continuous1.ArmArrives_Finish : [Sensors_80.O_80_Arm_Mag == true && ...
        | Status2b_15 == true]
    Distribution_Continuous1.PartDel_CheckLoop -> Distribution_Continuous1.ArmToMagazine1 [order 2] : [LoopDistCont == false]
    (junction 1736) -> Distribution_Continuous1.ArmArrives_FeedsPart
    (junction 1746) -> (junction 1736)
    Distribution_Continuous1.PartDel_CheckLoop -> (junction 1757) [order 1] : [LoopDistCont == true]
    Distribution_Continuous1.PartDel_CheckLoop -> Distribution_Continuous1.T1 [order 3] : after(4,sec)
    (junction 1757) -> (junction 1746)
  state Retrieve Part
    state FinishesProcess
      entry:
      Status5_13 = false;
      during:
      Control_90.C_95_PD_Proc;
      if Control_90.C_95_PD_Proc
      Status5_13 = true;
      else
      Status5_13 = false;
      end
    state InitialCondition
      entry:
      Status5_1 = false;
      during:
      AS_i_90.A_94_Cart_Full;
      Control_90.C_95_Initialization;
      Control_90.C_95_Cart2Del;
      Control_90.C_92_Profibus;
      Sensors_90.O_91_Key_Pos;
      if AS_i_90.A_94_Cart_Full && ...
      Control_90.C_95_Initialization && ...
      Control_90.C_95_Cart2Del && ...
      Control_90.C_92_Profibus && ...
      Sensors_90.O_91_Key_Pos
      Status5_1 = true;
      else
      Status5_1 = false;
      end
    (default) -> Retrieve.InitialCondition
    Retrieve.InitialCondition -> ? : [AS_i_90.A_94_CRoute_In == true && ...
        |  Status5_1 == true]
  state Distribution_Counted1
    state ArmToMagazine1
      entry:
      Status2c_14 = false;
      during:
      Actuators_80.F_82_Suction_Off;
      Actuators_80.F_82_Arm_2_Mag;
      Actuators_80.F_83_Led_Extra1;
      Control_80.C_85_Part_Del;
      if ~Actuators_80.F_82_Suction_Off && ...
      Actuators_80.F_82_Arm_2_Mag && ...
      Actuators_80.F_83_Led_Extra1 && ...
      Control_80.C_85_Part_Del
      Status2c_14 = true;
      else
      Status2c_14 = false;
      end
    state ArmCloseDeliver3
      entry:
      Status2c_15 = false;
      during:
      Sensors_70.O_70_SStation;
      if Sensors_70.O_70_SStation
      Status2c_15 = true;
      else
      Status2c_15 = false;
      end
    state ArmArrives_Finish
      entry:
      Status2c_16 = false;
      during:
      Actuators_80.F_82_Arm_2_Mag;
      if ~Actuators_80.F_82_Arm_2_Mag;
      Status2c_16 = true;
      else
      Status2c_16 = false;
      end
    state ArmToMagazine
      entry:
      Status2c_8 = false;
      during:
      Actuators_80.F_82_Arm_2_Mag;
      if Actuators_80.F_82_Arm_2_Mag
      Status2c_8 = true;
      else
      Status2c_8 = false;
      end
    state ArmCloseDeliver1
      entry:
      Status2c_9 = false;
      during:
      Sensors_70.O_70_SStation;
      if Sensors_70.O_70_SStation
      Status2c_9 = true;
      else
      Status2c_9 = false;
      end
    state ArmArrives_PicksPart
      entry:
      Status2c_10 = false;
      during:
      Actuators_80.F_82_Suction_On;
      Actuators_80.F_82_Arm_2_Mag;
